simulink model "Batbot_SIM"  (Simulink 7.5)
settings: Solver=ode45  StartTime=0.0  StopTime=5  FixedStep=0.1  RelTol=1e-3
values from neighbouring files (symbols this model uses):
  F_flapping = 1000    [SimulationFB.m]
  step_2 = tf/(col-1)    [SimulationFB.m]    (also in inverse_kinematicsFULLFB.m = 0.0114285714286)
libraries: mblibv1 x76, motdrv_lib x8, simulink x7
(part 2 of 3)

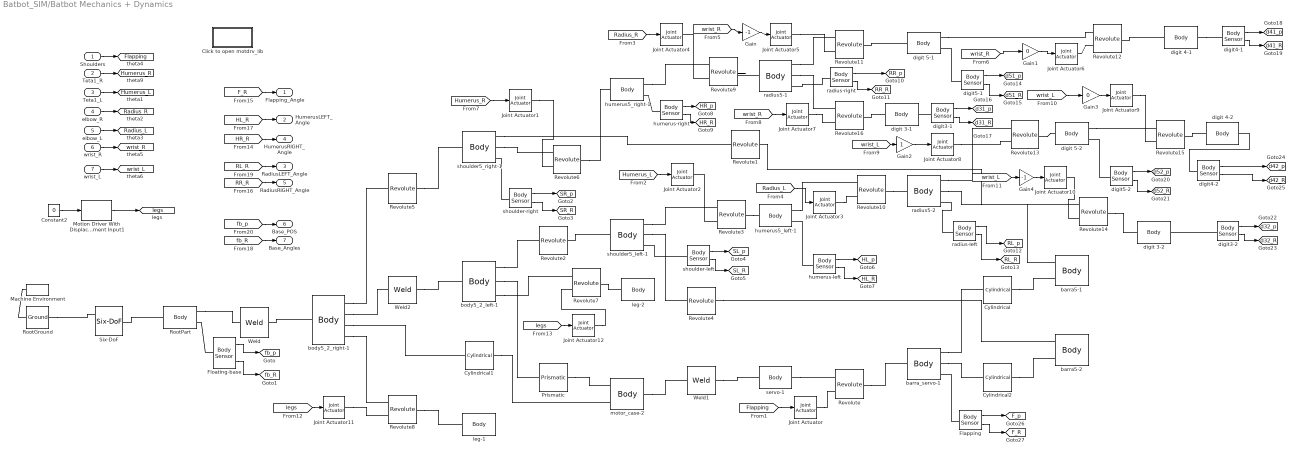
== system Batbot_SIM/Batbot Mechanics + Dynamics ==
  Shoulders : Inport  OutDataType=fixdt(1, 16)  OutScaling=2^0
  Teta1_R : Inport  Port=2  OutDataType=fixdt(1, 16)  OutScaling=2^0
  Teta1_L : Inport  Port=3  OutDataType=fixdt(1, 16)  OutScaling=2^0
  elbow_R : Inport  Port=4  OutDataType=fixdt(1, 16)  OutScaling=2^0
  elbow_L : Inport  Port=5  OutDataType=fixdt(1, 16)  OutScaling=2^0
  wrist_R : Inport  Port=6  OutDataType=fixdt(1, 16)  OutScaling=2^0
  wrist_L : Inport  Port=7  OutDataType=fixdt(1, 16)  OutScaling=2^0
  Click to open motdrv_lib : Subsystem
      settings: OpenFcn=open_system('motdrv_lib');
      mask Type: Double-click to open motdrv_lib
      mask Display: disp('motdrv_lib');
  Constant2 : Constant  Value=0  OutDataType=fixdt(1, 16)  OutScaling=2^0
  Cylindrical : mblibv1/Joints/Cylindrical  DialogController=MECH.DynMechDlgSource  PhysicalDomain=mechanical  SubClassName=Unknown  LeftPortType=blob  RightPortType=blob  LConnTagsString=__newl0  RConnTagsString=__newr0  UpdateFromCAD=on  NumSAPorts=0  CutJoint=off  MarkAsCut=off  Primitives=prismatic  PrimitiveProps=P1$WORLD$[0,0,1]$prismatic#R1$WORLD$[0,0,-1]$revolute  DialogClass=JointBlock  P1Axis=[0,0,1]  R1Axis=[0,0,-1]
  Cylindrical1 : mblibv1/Joints/Cylindrical  DialogController=MECH.DynMechDlgSource  PhysicalDomain=mechanical  SubClassName=Unknown  LeftPortType=blob  RightPortType=blob  LConnTagsString=__newl0  RConnTagsString=__newr0  UpdateFromCAD=on  NumSAPorts=0  CutJoint=off  MarkAsCut=off  Primitives=prismatic  PrimitiveProps=P1$WORLD$[0,0,-1]$prismatic#R1$WORLD$[0,0,1]$revolute  DialogClass=JointBlock  P1Axis=[0,0,-1]  R1Axis=[0,0,1]
  Cylindrical2 : mblibv1/Joints/Cylindrical  DialogController=MECH.DynMechDlgSource  PhysicalDomain=mechanical  SubClassName=Unknown  LeftPortType=blob  RightPortType=blob  LConnTagsString=__newl0  RConnTagsString=__newr0  UpdateFromCAD=on  NumSAPorts=0  CutJoint=off  MarkAsCut=off  Primitives=prismatic  PrimitiveProps=P1$WORLD$[0,0,1]$prismatic#R1$WORLD$[0,0,-1]$revolute  DialogClass=JointBlock  P1Axis=[0,0,1]  R1Axis=[0,0,-1]
  Flapping : mblibv1/Sensors &  Actuators/Body Sensor  DialogController=MECH.DynMechDlgSource  SystemSampleTime=-1  UpdateFromCAD=off  PhysicalDomain=Mechanical  PortType=blob  Muxed=off  Pose=on  Angle=on  AngleUnits=deg  ArcVelocity=off  ArcVelocityUnits=deg/s  ArcAcceleration=off  ArcAccelerationUnits=deg/s^2  CoordPosition=on  CoordPositionUnits=m  Velocity=off  VelocityUnits=m/s  Acceleration=off  AccelerationUnits=m/s^2  Quaternion=on  QuaternionDT=off  QuaternionDDT=off  QuaternionUnits=off  OutputVector=[1]  ActiveIO=on  Width=12  DialogClass=MechanicalSensorBlock  ReferenceFrame=Local (Body CS)
  Floating-base : mblibv1/Sensors &  Actuators/Body Sensor  DialogController=MECH.DynMechDlgSource  SystemSampleTime=-1  UpdateFromCAD=off  PhysicalDomain=Mechanical  PortType=blob  Muxed=off  Pose=on  Angle=on  AngleUnits=deg  ArcVelocity=off  ArcVelocityUnits=deg/s  ArcAcceleration=off  ArcAccelerationUnits=deg/s^2  CoordPosition=on  CoordPositionUnits=m  Velocity=off  VelocityUnits=m/s  Acceleration=off  AccelerationUnits=m/s^2  Quaternion=on  QuaternionDT=off  QuaternionDDT=off  QuaternionUnits=off  OutputVector=[1]  ActiveIO=on  Width=12  DialogClass=MechanicalSensorBlock  ReferenceFrame=Absolute (World)
  Gain : Gain  Gain=-1  ParameterDataType=fixdt(1, 16)  ParameterScaling=2^0  OutDataType=fixdt(1, 16)  OutScaling=2^0
  Gain1 : Gain  Gain=0  ParameterDataType=fixdt(1, 16)  ParameterScaling=2^0  OutDataType=fixdt(1, 16)  OutScaling=2^0
  Gain2 : Gain  ParameterDataType=fixdt(1, 16)  ParameterScaling=2^0  OutDataType=fixdt(1, 16)  OutScaling=2^0
  Gain3 : Gain  Gain=0  ParameterDataType=fixdt(1, 16)  ParameterScaling=2^0  OutDataType=fixdt(1, 16)  OutScaling=2^0
  Gain4 : Gain  Gain=-1  ParameterDataType=fixdt(1, 16)  ParameterScaling=2^0  OutDataType=fixdt(1, 16)  OutScaling=2^0
  Joint Actuator{,1..12} (13 alike) : mblibv1/Sensors &  Actuators/Joint Actuator  DialogController=MECH.DynMechDlgSource  SystemSampleTime=-1  UpdateFromCAD=off  PhysicalDomain=Mechanical  PortType=blob  ActuationStyle=Motion  AngleUnits=deg  ArcVelocityUnits=deg/s  ArcAccelerationUnits=deg/s^2  CoordPositionUnits=m  VelocityUnits=m/s  AccelerationUnits=m/s^2  ForceUnits=N  TorqueUnits=N*m  ActiveIO=on  Width=3  DialogClass=MechanicalActuatorBlock  Primitive=R1  ReferenceFrame=Absolute (World)
      settings: AttributesFormatString=ActuationStyle=%<ActuationStyle>
  Machine Environment : mblibv1/Bodies/Machine Environment  DialogController=MECH.DialogSource  SystemSampleTime=-1  PortType=env  PhysicalDomain=Mechanical  DialogTemplateClass=MECH.MachineEnvironment  SyncWhenCopied=off  Gravity=[0 0 0]  GravityUnits=m/s^2  GravityAsSignal=off  Dimensionality=Auto-detect  AnalysisType=Forward dynamics  LinearAssemblyTolerance=1e-3  LinearAssemblyToleranceUnits=m  AngularAssemblyTolerance=1e-3  AngularAssemblyToleranceUnits=rad  ConstraintSolverType=Stabilizing  ConstraintRelTolerance=1e-4  ConstraintAbsTolerance=1e-4  UseRobustSingularityHandling=off  RedundancyAnalysisToleranceType=Automatically select tolerance  RedundancyAnalysisTolerance=1e-14  StatePerturbationType=Fixed  PerturbationSize=1e-5  VisualizeMachine=on  BodyVisualizationType=Use model default body geometries  BodyColorSelMode=Use model default  DefaultBodyColor=[1 0 0]
  Motion Driver With Displacement Input1 : motdrv_lib/Motion Driver With Displacement Input  SystemSampleTime=-1  InitialDisplacementSource=Dialog  InitialDisplacement=0  InitialVelocity=0  TimeConstant=1e-3
  Prismatic : mblibv1/Joints/Prismatic  DialogController=MECH.DynMechDlgSource  PhysicalDomain=mechanical  SubClassName=Unknown  LeftPortType=blob  RightPortType=blob  LConnTagsString=__newl0  RConnTagsString=__newr0  UpdateFromCAD=on  NumSAPorts=0  CutJoint=off  MarkAsCut=off  Primitives=prismatic  PrimitiveProps=P1$WORLD$[-1,0,0]$prismatic  DialogClass=JointBlock  P1Axis=[-1,0,0]
  Revolute : mblibv1/Joints/Revolute  DialogController=MECH.DynMechDlgSource  PhysicalDomain=mechanical  SubClassName=Unknown  LeftPortType=blob  RightPortType=blob  LConnTagsString=__newl0|SA1  RConnTagsString=__newr0  UpdateFromCAD=on  NumSAPorts=1  CutJoint=off  MarkAsCut=off  Primitives=prismatic  PrimitiveProps=R1$Base$[0,0,-1]$revolute  DialogClass=JointBlock  R1Axis=[0,0,-1]
  Revolute1 : mblibv1/Joints/Revolute  DialogController=MECH.DynMechDlgSource  PhysicalDomain=mechanical  SubClassName=Unknown  LeftPortType=blob  RightPortType=blob  LConnTagsString=__newl0  RConnTagsString=__newr0  UpdateFromCAD=on  NumSAPorts=0  CutJoint=off  MarkAsCut=off  Primitives=prismatic  PrimitiveProps=R1$WORLD$[0,0,-1]$revolute  DialogClass=JointBlock  R1Axis=[0,0,-1]
  Revolute10 : mblibv1/Joints/Revolute  DialogController=MECH.DynMechDlgSource  PhysicalDomain=mechanical  SubClassName=Unknown  LeftPortType=blob  RightPortType=blob  LConnTagsString=__newl0|SA1  RConnTagsString=__newr0  UpdateFromCAD=on  NumSAPorts=1  CutJoint=off  MarkAsCut=off  Primitives=prismatic  PrimitiveProps=R1$Base$[0.343768,-0.939055,0]$revolute  DialogClass=JointBlock  R1Axis=[0.343768,-0.939055,0]
  Revolute11 : mblibv1/Joints/Revolute  DialogController=MECH.DynMechDlgSource  PhysicalDomain=mechanical  SubClassName=Unknown  LeftPortType=blob  RightPortType=blob  LConnTagsString=__newl0|SA1  RConnTagsString=__newr0  UpdateFromCAD=on  NumSAPorts=1  CutJoint=off  MarkAsCut=off  Primitives=prismatic  PrimitiveProps=R1$Base$[-0.399458,-0.916751,0]$revolute  DialogClass=JointBlock  R1Axis=[-0.399458,-0.916751,0]
  Revolute12 : mblibv1/Joints/Revolute  DialogController=MECH.DynMechDlgSource  PhysicalDomain=mechanical  SubClassName=Unknown  LeftPortType=blob  RightPortType=blob  LConnTagsString=__newl0|SA1  RConnTagsString=__newr0  UpdateFromCAD=on  NumSAPorts=1  CutJoint=off  MarkAsCut=off  Primitives=prismatic  PrimitiveProps=R1$Base$[0.399458,0.916751,0]$revolute  DialogClass=JointBlock  R1Axis=[0.399458,0.916751,0]
  Revolute13 : mblibv1/Joints/Revolute  DialogController=MECH.DynMechDlgSource  PhysicalDomain=mechanical  SubClassName=Unknown  LeftPortType=blob  RightPortType=blob  LConnTagsString=__newl0|SA1  RConnTagsString=__newr0  UpdateFromCAD=on  NumSAPorts=1  CutJoint=off  MarkAsCut=off  Primitives=prismatic  PrimitiveProps=R1$Base$[-0.343768,0.939055,0]$revolute  DialogClass=JointBlock  R1Axis=[-0.343768,0.939055,0]
  Revolute14 : mblibv1/Joints/Revolute  DialogController=MECH.DynMechDlgSource  PhysicalDomain=mechanical  SubClassName=Unknown  LeftPortType=blob  RightPortType=blob  LConnTagsString=__newl0|SA1  RConnTagsString=__newr0  UpdateFromCAD=on  NumSAPorts=1  CutJoint=off  MarkAsCut=off  Primitives=prismatic  PrimitiveProps=R1$Base$[0.343768,-0.939055,0]$revolute  DialogClass=JointBlock  R1Axis=[0.343768,-0.939055,0]
  Revolute15 : mblibv1/Joints/Revolute  DialogController=MECH.DynMechDlgSource  PhysicalDomain=mechanical  SubClassName=Unknown  LeftPortType=blob  RightPortType=blob  LConnTagsString=__newl0|SA1  RConnTagsString=__newr0  UpdateFromCAD=on  NumSAPorts=1  CutJoint=off  MarkAsCut=off  Primitives=prismatic  PrimitiveProps=R1$Base$[-0.343768,0.939055,0]$revolute  DialogClass=JointBlock  R1Axis=[-0.343768,0.939055,0]
  Revolute16 : mblibv1/Joints/Revolute  DialogController=MECH.DynMechDlgSource  PhysicalDomain=mechanical  SubClassName=Unknown  LeftPortType=blob  RightPortType=blob  LConnTagsString=__newl0|SA1  RConnTagsString=__newr0  UpdateFromCAD=on  NumSAPorts=1  CutJoint=off  MarkAsCut=off  Primitives=prismatic  PrimitiveProps=R1$Base$[0.399458,0.916751,0]$revolute  DialogClass=JointBlock  R1Axis=[0.399458,0.916751,0]
  Revolute2 : mblibv1/Joints/Revolute  DialogController=MECH.DynMechDlgSource  PhysicalDomain=mechanical  SubClassName=Unknown  LeftPortType=blob  RightPortType=blob  LConnTagsString=__newl0  RConnTagsString=__newr0  UpdateFromCAD=on  NumSAPorts=0  CutJoint=off  MarkAsCut=off  Primitives=prismatic  PrimitiveProps=R1$World$[0,0,-1]$revolute  DialogClass=JointBlock  R1Axis=[0,0,-1]
  Revolute3 : mblibv1/Joints/Revolute  DialogController=MECH.DynMechDlgSource  PhysicalDomain=mechanical  SubClassName=Unknown  LeftPortType=blob  RightPortType=blob  LConnTagsString=__newl0|SA1  RConnTagsString=__newr0  UpdateFromCAD=on  NumSAPorts=1  CutJoint=off  MarkAsCut=off  Primitives=prismatic  PrimitiveProps=R1$Base$[0.343768,-0.939055,0]$revolute  DialogClass=JointBlock  R1Axis=[0.343768,-0.939055,0]
  Revolute4 : mblibv1/Joints/Revolute  DialogController=MECH.DynMechDlgSource  PhysicalDomain=mechanical  SubClassName=Unknown  LeftPortType=blob  RightPortType=blob  LConnTagsString=__newl0  RConnTagsString=__newr0  UpdateFromCAD=on  NumSAPorts=0  CutJoint=off  MarkAsCut=off  Primitives=prismatic  PrimitiveProps=R1$WORLD$[0,0,-1]$revolute  DialogClass=JointBlock  R1Axis=[0,0,-1]
  Revolute5 : mblibv1/Joints/Revolute  DialogController=MECH.DynMechDlgSource  PhysicalDomain=mechanical  SubClassName=Unknown  LeftPortType=blob  RightPortType=blob  LConnTagsString=__newl0  RConnTagsString=__newr0  UpdateFromCAD=on  NumSAPorts=0  CutJoint=off  MarkAsCut=off  Primitives=prismatic  PrimitiveProps=R1$World$[0,0,1]$revolute  DialogClass=JointBlock  R1Axis=[0,0,1]
  Revolute6 : mblibv1/Joints/Revolute  DialogController=MECH.DynMechDlgSource  PhysicalDomain=mechanical  SubClassName=Unknown  LeftPortType=blob  RightPortType=blob  LConnTagsString=__newl0|SA1  RConnTagsString=__newr0  UpdateFromCAD=on  NumSAPorts=1  CutJoint=off  MarkAsCut=off  Primitives=prismatic  PrimitiveProps=R1$Base$[0.399458,0.916751,0]$revolute  DialogClass=JointBlock  R1Axis=[0.399458,0.916751,0]
  Revolute7 : mblibv1/Joints/Revolute  DialogController=MECH.DynMechDlgSource  PhysicalDomain=mechanical  SubClassName=Unknown  LeftPortType=blob  RightPortType=blob  LConnTagsString=__newl0|SA1  RConnTagsString=__newr0  UpdateFromCAD=on  NumSAPorts=1  CutJoint=off  MarkAsCut=off  Primitives=prismatic  PrimitiveProps=R1$Base$[0,1,0]$revolute  DialogClass=JointBlock  R1Axis=[0,1,0]
  Revolute8 : mblibv1/Joints/Revolute  DialogController=MECH.DynMechDlgSource  PhysicalDomain=mechanical  SubClassName=Unknown  LeftPortType=blob  RightPortType=blob  LConnTagsString=__newl0|SA1  RConnTagsString=__newr0  UpdateFromCAD=on  NumSAPorts=1  CutJoint=off  MarkAsCut=off  Primitives=prismatic  PrimitiveProps=R1$Base$[0,-1,0]$revolute  DialogClass=JointBlock  R1Axis=[0,-1,0]
  Revolute9 : mblibv1/Joints/Revolute  DialogController=MECH.DynMechDlgSource  PhysicalDomain=mechanical  SubClassName=Unknown  LeftPortType=blob  RightPortType=blob  LConnTagsString=__newl0|SA1  RConnTagsString=__newr0  UpdateFromCAD=on  NumSAPorts=1  CutJoint=off  MarkAsCut=off  Primitives=prismatic  PrimitiveProps=R1$Base$[-0.399458,-0.916751,0]$revolute  DialogClass=JointBlock  R1Axis=[-0.399458,-0.916751,0]
  RootGround : mblibv1/Bodies/Ground  DialogController=MECH.DynMechDlgSource  SystemSampleTime=-1  UpdateFromCAD=on  LeftPortType=env  RightPortType=workingframe  PhysicalDomain=Mechanical  DialogClass=GroundBlock  CoordPosition=[-0.0126203,-0.00464218,0.00877209]  CoordPositionUnits=m  StateVectorMgrId=0  MachineId=[1 0]  ShowEnvPort=on
  RootPart : mblibv1/Bodies/Body  DialogController=MECH.DynMechDlgSource  PhysicalDomain=mechanical  SubClassName=Unknown  LeftPortType=workingframe  RightPortType=workingframe  LConnTagsString=CS3  RConnTagsString=CS2|CS1  UpdateFromCAD=on  DialogClass=MechanicalBodyBlock  Mass=0  MassUnits=kg  InertiaUnits=kg*m^2  Inertia=[0,0,0;0,0,0;0,0,0]  Shape=Cylinder  ShapeDims=[1 1]  ShapeUnits=m  ShapeUse=false  Density=1  DensityUnits=kg/m^3  DensityUse=false  GraphicsMode=MACHINE_DEFAULT  BodyColorSelMode=MACHINE_DEFAULT  BodyColor=[1 0 0]  AttachedToCS=CS1  CG=Right$CG$[-0.0126203 -0.00464218 0.00877209]$WORLD$WORLD$m$[1 0 0;0 1 0;0 0 1]$3x3 Transform$rad$WORLD$false$none  WorkingFrames=Right$CS2$[0.0103788 -0.00702282 0.00503904]$WORLD$WORLD$m$[1 0 0;0 1 0;0 0 1]$3x3 Transform$rad$WORLD$true$none#Left$CS3$[-0.0126203 -0.00464218 0.00877209]$WORLD$WORLD$m$[1 0 0;0 1 0;0 0 1]$3x3 Transform$rad$WORLD$true$none#Right$CS1$[0 0 0]$WORLD$WORLD$m$[1 0 0;0 1 0;0 0 1]$3x3 Transform$rad$WORLD$true$none  CGPos=[-0.0126203 -0.00464218 0.00877209]  CGRot=[1 0 0;0 1 0;0 0 1]  CS0Pos=[]  CS0Rot=[]  CS1Pos=[0 0 0]  CS1Rot=[1 0 0;0 1 0;0 0 1]  CS2Pos=[0.0103788 -0.00702282 0.00503904]  CS2Rot=[1 0 0;0 1 0;0 0 1]  CS3Pos=[-0.0126203 -0.00464218 0.00877209]  CS3Rot=[1 0 0;0 1 0;0 0 1]  CS4Pos=[]  CS4Rot=[]  CS5Pos=[]  CS5Rot=[]  CS6Pos=[]  CS6Rot=[]  CS7Pos=[]  CS7Rot=[]  CS8Pos=[]  CS8Rot=[]  CS9Pos=[]  CS9Rot=[]  CS10Pos=[]  CS10Rot=[]  CS11Pos=[]  CS11Rot=[]  CS12Pos=[]  CS12Rot=[]  CS13Pos=[]  CS13Rot=[]  CS14Pos=[]  CS14Rot=[]  CS15Pos=[]  CS15Rot=[]  CS16Pos=[]  CS16Rot=[]  CS17Pos=[]  CS17Rot=[]  CS18Pos=[]  CS18Rot=[]  CS19Pos=[]  CS19Rot=[]  CS20Pos=[]  CS20Rot=[]
  Six-DoF : mblibv1/Joints/Six-DoF  DialogController=MECH.DynMechDlgSource  PhysicalDomain=mechanical  SubClassName=Unknown  LeftPortType=blob  RightPortType=blob  LConnTagsString=__newl0|SA1  RConnTagsString=__newr0  UpdateFromCAD=off  NumSAPorts=1  CutJoint=off  MarkAsCut=off  Primitives=prismatic_prismatic  PrimitiveProps=P1$World$[1 0 0]$prismatic#P2$World$[0 1 0]$prismatic#P3$World$[0 0 1]$prismatic#S$World$[0 0 0]$spherical  DialogClass=JointBlock  P1Axis=[1 0 0]  P2Axis=[0 1 0]  P3Axis=[0 0 1]  SAxis=[0 0 0]
  Weld : mblibv1/Joints/Weld  DialogController=MECH.DynMechDlgSource  PhysicalDomain=mechanical  SubClassName=Unknown  LeftPortType=blob  RightPortType=blob  LConnTagsString=__newl0  RConnTagsString=__newr0  UpdateFromCAD=on  NumSAPorts=0  CutJoint=off  MarkAsCut=off  Primitives=weld  PrimitiveProps=W$World$[0.57735,0.57735,0.57735]$weld  DialogClass=JointBlock  WAxis=[0.57735,0.57735,0.57735]
  Weld1 : mblibv1/Joints/Weld  DialogController=MECH.DynMechDlgSource  PhysicalDomain=mechanical  SubClassName=Unknown  LeftPortType=blob  RightPortType=blob  LConnTagsString=__newl0  RConnTagsString=__newr0  UpdateFromCAD=on  NumSAPorts=0  CutJoint=off  MarkAsCut=off  Primitives=weld  PrimitiveProps=W$WORLD$[0.57735,0.57735,0.57735]$weld  DialogClass=JointBlock  WAxis=[0.57735,0.57735,0.57735]
  Weld2 : mblibv1/Joints/Weld  DialogController=MECH.DynMechDlgSource  PhysicalDomain=mechanical  SubClassName=Unknown  LeftPortType=blob  RightPortType=blob  LConnTagsString=__newl0  RConnTagsString=__newr0  UpdateFromCAD=on  NumSAPorts=0  CutJoint=off  MarkAsCut=off  Primitives=weld  PrimitiveProps=W$WORLD$[0.57735,0.57735,0.57735]$weld  DialogClass=JointBlock  WAxis=[0.57735,0.57735,0.57735]
  barra5-1 : mblibv1/Bodies/Body  DialogController=MECH.DynMechDlgSource  PhysicalDomain=mechanical  SubClassName=Unknown  LeftPortType=workingframe  RightPortType=workingframe  LConnTagsString=CS2|CS3  UpdateFromCAD=on  DialogClass=MechanicalBodyBlock  Mass=0.000119962  MassUnits=kg  InertiaUnits=kg*m^2  Inertia=[1.1412e-010,-3.7491e-012,4.37309e-017;-3.7491e-012,8.63077e-009,-5.97977e-019;4.37309e-017,-5.97977e-019,8.66519e-009]  Shape=Cylinder  ShapeDims=[1 1]  ShapeUnits=m  ShapeUse=false  Density=1  DensityUnits=kg/m^3  DensityUse=false  GraphicsMode=GFXFILE  GraphicsFileName=Batbot - barra5-1.STL  BodyColorSelMode=COLORPALETTE  BodyColor=[0.25098 0.25098 0.25098]  AttachedToCS=CS1  CG=Right$CG$[0.00675046 0.021022 0.006]$WORLD$WORLD$m$[0.97857 0.205912 0;-0.205912 0.97857 0;0 0 1]$3x3 Transform$rad$WORLD$false$none  WorkingFrames=Right$CS1$[-0.00713958 0.0218999 0.007]$WORLD$WORLD$m$[0.97857 0.205912 0;-0.205912 0.97857 0;0 0 1]$3x3 Transform$rad$WORLD$false$none#Left$CS2$[0.0201957 0.0181917 0.005]$WORLD$WORLD$m$[1 0 0;0 1 0;0 0 1]$3x3 Transform$rad$WORLD$true$none#Left$CS3$[-0.00672776 0.023857 0.005]$WORLD$WORLD$m$[1 0 0;0 1 0;0 0 1]$3x3 Transform$rad$WORLD$true$none#Right$CS4$[0 0 0]$WORLD$WORLD$m$[1 0 0;0 1 0;0 0 1]$3x3 Transform$rad$WORLD$false$none  CGPos=[0.00675046 0.021022 0.006]  CGRot=[0.97857 0.205912 0;-0.205912 0.97857 0;0 0 1]  CS0Pos=[]  CS0Rot=[]  CS1Pos=[-0.00713958 0.0218999 0.007]  CS1Rot=[0.97857 0.205912 0;-0.205912 0.97857 0;0 0 1]  CS2Pos=[0.0201957 0.0181917 0.005]  CS2Rot=[1 0 0;0 1 0;0 0 1]  CS3Pos=[-0.00672776 0.023857 0.005]  CS3Rot=[1 0 0;0 1 0;0 0 1]  CS4Pos=[0 0 0]  CS4Rot=[1 0 0;0 1 0;0 0 1]  CS5Pos=[]  CS5Rot=[]  CS6Pos=[]  CS6Rot=[]  CS7Pos=[]  CS7Rot=[]  CS8Pos=[]  CS8Rot=[]  CS9Pos=[]  CS9Rot=[]  CS10Pos=[]  CS10Rot=[]  CS11Pos=[]  CS11Rot=[]  CS12Pos=[]  CS12Rot=[]  CS13Pos=[]  CS13Rot=[]  CS14Pos=[]  CS14Rot=[]  CS15Pos=[]  CS15Rot=[]  CS16Pos=[]  CS16Rot=[]  CS17Pos=[]  CS17Rot=[]  CS18Pos=[]  CS18Rot=[]  CS19Pos=[]  CS19Rot=[]  CS20Pos=[]  CS20Rot=[]
  barra5-2 : mblibv1/Bodies/Body  DialogController=MECH.DynMechDlgSource  PhysicalDomain=mechanical  SubClassName=Unknown  LeftPortType=workingframe  RightPortType=workingframe  LConnTagsString=CS2|CS3  UpdateFromCAD=on  DialogClass=MechanicalBodyBlock  Mass=0.000119962  MassUnits=kg  InertiaUnits=kg*m^2  Inertia=[1.1412e-010,-3.7491e-012,4.37309e-017;-3.7491e-012,8.63077e-009,-5.97977e-019;4.37309e-017,-5.97977e-019,8.66519e-009]  Shape=Cylinder  ShapeDims=[1 1]  ShapeUnits=m  ShapeUse=false  Density=1  DensityUnits=kg/m^3  DensityUse=false  GraphicsMode=GFXFILE  GraphicsFileName=Batbot - barra5-2.STL  BodyColorSelMode=COLORPALETTE  BodyColor=[0.25098;0.25098;0.25098]  AttachedToCS=CS1  CG=Right$CG$[-0.0314187 0.0149284 0.006]$WORLD$WORLD$m$[0.96422 0.265104 0;-0.265104 0.96422 0;0 0 1]$3x3 Transform$rad$WORLD$false$none  WorkingFrames=Right$CS1$[-0.0452295 0.0166503 0.007]$WORLD$WORLD$m$[0.96422 0.265104 0;-0.265104 0.96422 0;0 0 1]$3x3 Transform$rad$WORLD$false$none#Left$CS2$[-0.0446993 0.0185787 0.005]$WORLD$WORLD$m$[1 0 0;0 1 0;0 0 1]$3x3 Transform$rad$WORLD$true$none#Left$CS3$[-0.0181707 0.0112849 0.005]$WORLD$WORLD$m$[1 0 0;0 1 0;0 0 1]$3x3 Transform$rad$WORLD$true$none  CGPos=[-0.0314187 0.0149284 0.006]  CGRot=[0.96422 0.265104 0;-0.265104 0.96422 0;0 0 1]  CS0Pos=[]  CS0Rot=[]  CS1Pos=[-0.0452295 0.0166503 0.007]  CS1Rot=[0.96422 0.265104 0;-0.265104 0.96422 0;0 0 1]  CS2Pos=[-0.0446993 0.0185787 0.005]  CS2Rot=[1 0 0;0 1 0;0 0 1]  CS3Pos=[-0.0181707 0.0112849 0.005]  CS3Rot=[1 0 0;0 1 0;0 0 1]  CS4Pos=[]  CS4Rot=[]  CS5Pos=[]  CS5Rot=[]  CS6Pos=[]  CS6Rot=[]  CS7Pos=[]  CS7Rot=[]  CS8Pos=[]  CS8Rot=[]  CS9Pos=[]  CS9Rot=[]  CS10Pos=[]  CS10Rot=[]  CS11Pos=[]  CS11Rot=[]  CS12Pos=[]  CS12Rot=[]  CS13Pos=[]  CS13Rot=[]  CS14Pos=[]  CS14Rot=[]  CS15Pos=[]  CS15Rot=[]  CS16Pos=[]  CS16Rot=[]  CS17Pos=[]  CS17Rot=[]  CS18Pos=[]  CS18Rot=[]  CS19Pos=[]  CS19Rot=[]  CS20Pos=[]  CS20Rot=[]
  barra_servo-1 : mblibv1/Bodies/Body  DialogController=MECH.DynMechDlgSource  PhysicalDomain=mechanical  SubClassName=Unknown  LeftPortType=workingframe  RightPortType=workingframe  LConnTagsString=CS2  RConnTagsString=CS3|CS4|CS5  UpdateFromCAD=on  DialogClass=MechanicalBodyBlock  Mass=0.00014427  MassUnits=kg  InertiaUnits=kg*m^2  Inertia=[7.38605e-009,0,0;0,7.70092e-009,0;0,0,5.0296e-010]  Shape=Cylinder  ShapeDims=[1 1]  ShapeUnits=m  ShapeUse=false  Density=1  DensityUnits=kg/m^3  DensityUse=false  GraphicsMode=GFXFILE  GraphicsFileName=Batbot - barra_servo-1.STL  BodyColorSelMode=COLORPALETTE  BodyColor=[1 1 1]  AttachedToCS=CS1  CG=Right$CG$[-0.0124493 0.017571 0.00472003]$WORLD$WORLD$m$[-0.739536 0 -0.673117;0.673117 0 -0.739536;0 -1 0]$3x3 Transform$rad$WORLD$false$none  WorkingFrames=Right$CS1$[-0.0124493 0.017571 0.0095]$WORLD$WORLD$m$[-0.739536 0 -0.673117;0.673117 0 -0.739536;0 -1 0]$3x3 Transform$rad$WORLD$false$none#Left$CS2$[-0.0124493 0.017571 0.0095]$WORLD$WORLD$m$[1 0 0;0 1 0;0 0 1]$3x3 Transform$rad$WORLD$true$none#Right$CS3$[-0.00672776 0.023857 0.005]$WORLD$WORLD$m$[1 0 0;0 1 0;0 0 1]$3x3 Transform$rad$WORLD$true$none#Right$CS4$[-0.0181707 0.0112849 0.005]$WORLD$WORLD$m$[1 0 0;0 1 0;0 0 1]$3x3 Transform$rad$WORLD$true$none#Right$CS5$[0 0 0]$WORLD$WORLD$m$[1 0 0;0 1 0;0 0 1]$3x3 Transform$rad$WORLD$true$none  CGPos=[-0.0124493 0.017571 0.00472003]  CGRot=[-0.739536 0 -0.673117;0.673117 0 -0.739536;0 -1 0]  CS0Pos=[]  CS0Rot=[]  CS1Pos=[-0.0124493 0.017571 0.0095]  CS1Rot=[-0.739536 0 -0.673117;0.673117 0 -0.739536;0 -1 0]  CS2Pos=[-0.0124493 0.017571 0.0095]  CS2Rot=[1 0 0;0 1 0;0 0 1]  CS3Pos=[-0.00672776 0.023857 0.005]  CS3Rot=[1 0 0;0 1 0;0 0 1]  CS4Pos=[-0.0181707 0.0112849 0.005]  CS4Rot=[1 0 0;0 1 0;0 0 1]  CS5Pos=[0 0 0]  CS5Rot=[1 0 0;0 1 0;0 0 1]  CS6Pos=[]  CS6Rot=[]  CS7Pos=[]  CS7Rot=[]  CS8Pos=[]  CS8Rot=[]  CS9Pos=[]  CS9Rot=[]  CS10Pos=[]  CS10Rot=[]  CS11Pos=[]  CS11Rot=[]  CS12Pos=[]  CS12Rot=[]  CS13Pos=[]  CS13Rot=[]  CS14Pos=[]  CS14Rot=[]  CS15Pos=[]  CS15Rot=[]  CS16Pos=[]  CS16Rot=[]  CS17Pos=[]  CS17Rot=[]  CS18Pos=[]  CS18Rot=[]  CS19Pos=[]  CS19Rot=[]  CS20Pos=[]  CS20Rot=[]
  body5_2_left-1 : mblibv1/Bodies/Body  DialogController=MECH.DynMechDlgSource  PhysicalDomain=mechanical  SubClassName=Unknown  LeftPortType=workingframe  RightPortType=workingframe  LConnTagsString=CS3  RConnTagsString=CS2|CS4|CS5  UpdateFromCAD=on  DialogClass=MechanicalBodyBlock  Mass=0.00990124  MassUnits=kg  InertiaUnits=kg*m^2  Inertia=[6.86716e-006,1.97503e-007,-1.60321e-007;1.97503e-007,6.52126e-006,2.23269e-008;-1.60321e-007,2.23269e-008,1.26887e-006]  Shape=Cylinder  ShapeDims=[1 1]  ShapeUnits=m  ShapeUse=false  Density=1  DensityUnits=kg/m^3  DensityUse=false  GraphicsMode=GFXFILE  GraphicsFileName=Batbot - body5_2_left-1.STL  BodyColorSelMode=COLORPALETTE  BodyColor=[0.25098;0.25098;0.25098]  AttachedToCS=CS1  CG=Right$CG$[-0.0358488 -0.00702322 0.00503721]$WORLD$WORLD$m$[1 0 0;0 1 0;0 0 1]$3x3 Transform$rad$WORLD$false$none  WorkingFrames=Right$CS1$[0.00126505 0.00228611 -2.18436e-014]$WORLD$WORLD$m$[1 0 0;0 1 0;0 0 1]$3x3 Transform$rad$WORLD$false$none#Right$CS2$[-0.0387349 0.00228611 0.034]$WORLD$WORLD$m$[1 0 0;0 1 0;0 0 1]$3x3 Transform$rad$WORLD$true$none#Left$CS3$[-0.0127349 -0.0177139 0.035]$WORLD$WORLD$m$[1 0 0;0 1 0;0 0 1]$3x3 Transform$rad$WORLD$true$none#Right$CS4$[-0.0127349 -0.0167139 0.019]$WORLD$WORLD$m$[1 0 0;0 1 0;0 0 1]$3x3 Transform$rad$WORLD$true$none#Right$CS5$[-0.0367349 0.00438611 0.052]$WORLD$WORLD$m$[1 0 0;0 1 0;0 0 1]$3x3 Transform$rad$WORLD$true$none  CGPos=[-0.0358488 -0.00702322 0.00503721]  CGRot=[1 0 0;0 1 0;0 0 1]  CS0Pos=[]  CS0Rot=[]  CS1Pos=[0.00126505 0.00228611 -2.18436e-014]  CS1Rot=[1 0 0;0 1 0;0 0 1]  CS2Pos=[-0.0387349 0.00228611 0.034]  CS2Rot=[1 0 0;0 1 0;0 0 1]  CS3Pos=[-0.0127349 -0.0177139 0.035]  CS3Rot=[1 0 0;0 1 0;0 0 1]  CS4Pos=[-0.0127349 -0.0167139 0.019]  CS4Rot=[1 0 0;0 1 0;0 0 1]  CS5Pos=[-0.0367349 0.00438611 0.052]  CS5Rot=[1 0 0;0 1 0;0 0 1]  CS6Pos=[]  CS6Rot=[]  CS7Pos=[]  CS7Rot=[]  CS8Pos=[]  CS8Rot=[]  CS9Pos=[]  CS9Rot=[]  CS10Pos=[]  CS10Rot=[]  CS11Pos=[]  CS11Rot=[]  CS12Pos=[]  CS12Rot=[]  CS13Pos=[]  CS13Rot=[]  CS14Pos=[]  CS14Rot=[]  CS15Pos=[]  CS15Rot=[]  CS16Pos=[]  CS16Rot=[]  CS17Pos=[]  CS17Rot=[]  CS18Pos=[]  CS18Rot=[]  CS19Pos=[]  CS19Rot=[]  CS20Pos=[]  CS20Rot=[]
  body5_2_right-1 : mblibv1/Bodies/Body  DialogController=MECH.DynMechDlgSource  PhysicalDomain=mechanical  SubClassName=Unknown  LeftPortType=workingframe  RightPortType=workingframe  LConnTagsString=CS2  RConnTagsString=CS3|CS4|CS5|CS6  UpdateFromCAD=on  DialogClass=MechanicalBodyBlock  Mass=0.00990077  MassUnits=kg  InertiaUnits=kg*m^2  Inertia=[6.8671e-006,-1.97521e-007,1.60303e-007;-1.97521e-007,6.52112e-006,2.23345e-008;1.60303e-007,2.23345e-008,1.26891e-006]  Shape=Cylinder  ShapeDims=[1 1]  ShapeUnits=m  ShapeUse=false  Density=1  DensityUnits=kg/m^3  DensityUse=false  GraphicsMode=GFXFILE  GraphicsFileName=Batbot - body5_2_right-1.STL  BodyColorSelMode=COLORPALETTE  BodyColor=[0.25098;0.25098;0.25098]  AttachedToCS=CS1  CG=Right$CG$[0.0103788 -0.00702282 0.00503904]$WORLD$WORLD$m$[1 0 0;0 1 0;0 0 1]$3x3 Transform$rad$WORLD$false$none  WorkingFrames=Right$CS1$[0.00126505 0.00228611 -2.18402e-014]$WORLD$WORLD$m$[1 0 0;0 1 0;0 0 1]$3x3 Transform$rad$WORLD$false$none#Left$CS2$[0.0103788 -0.00702282 0.00503904]$WORLD$WORLD$m$[1 0 0;0 1 0;0 0 1]$3x3 Transform$rad$WORLD$true$none#Right$CS3$[0.0132651 0.00228611 0.034]$WORLD$WORLD$m$[1 0 0;0 1 0;0 0 1]$3x3 Transform$rad$WORLD$true$none#Right$CS4$[-0.0127349 -0.0177139 0.035]$WORLD$WORLD$m$[1 0 0;0 1 0;0 0 1]$3x3 Transform$rad$WORLD$true$none#Right$CS5$[-0.00498495 -0.0167139 0.019]$WORLD$WORLD$m$[1 0 0;0 1 0;0 0 1]$3x3 Transform$rad$WORLD$true$none#Right$CS6$[0.0112651 0.00438611 0.052]$WORLD$WORLD$m$[1 0 0;0 1 0;0 0 1]$3x3 Transform$rad$WORLD$true$none  CGPos=[0.0103788 -0.00702282 0.00503904]  CGRot=[1 0 0;0 1 0;0 0 1]  CS0Pos=[]  CS0Rot=[]  CS1Pos=[0.00126505 0.00228611 -2.18402e-014]  CS1Rot=[1 0 0;0 1 0;0 0 1]  CS2Pos=[0.0103788 -0.00702282 0.00503904]  CS2Rot=[1 0 0;0 1 0;0 0 1]  CS3Pos=[0.0132651 0.00228611 0.034]  CS3Rot=[1 0 0;0 1 0;0 0 1]  CS4Pos=[-0.0127349 -0.0177139 0.035]  CS4Rot=[1 0 0;0 1 0;0 0 1]  CS5Pos=[-0.00498495 -0.0167139 0.019]  CS5Rot=[1 0 0;0 1 0;0 0 1]  CS6Pos=[0.0112651 0.00438611 0.052]  CS6Rot=[1 0 0;0 1 0;0 0 1]  CS7Pos=[]  CS7Rot=[]  CS8Pos=[]  CS8Rot=[]  CS9Pos=[]  CS9Rot=[]  CS10Pos=[]  CS10Rot=[]  CS11Pos=[]  CS11Rot=[]  CS12Pos=[]  CS12Rot=[]  CS13Pos=[]  CS13Rot=[]  CS14Pos=[]  CS14Rot=[]  CS15Pos=[]  CS15Rot=[]  CS16Pos=[]  CS16Rot=[]  CS17Pos=[]  CS17Rot=[]  CS18Pos=[]  CS18Rot=[]  CS19Pos=[]  CS19Rot=[]  CS20Pos=[]  CS20Rot=[]
  digit 3-1 : mblibv1/Bodies/Body  DialogController=MECH.DynMechDlgSource  PhysicalDomain=mechanical  SubClassName=Unknown  LeftPortType=workingframe  RightPortType=workingframe  LConnTagsString=CS2  RConnTagsString=CS3  UpdateFromCAD=on  DialogClass=MechanicalBodyBlock  Mass=0.000927477  MassUnits=kg  InertiaUnits=kg*m^2  Inertia=[4.25859e-008,5.30437e-013,-1.56119e-007;5.30437e-013,9.99762e-007,1.56782e-013;-1.56119e-007,1.56782e-013,9.57517e-007]  Shape=Cylinder  ShapeDims=[1 1]  ShapeUnits=m  ShapeUse=false  Density=1  DensityUnits=kg/m^3  DensityUse=false  GraphicsMode=GFXFILE  GraphicsFileName=Batbot - digit 3-1.STL  BodyColorSelMode=COLORPALETTE  BodyColor=[0.25098 0.25098 0.25098]  AttachedToCS=CS1  CG=Right$CG$[0.133076 -0.047356 -0.0341214]$WORLD$WORLD$m$[0.916713 0.399458 0.0083752;-0.399442 0.916751 -0.00364935;-0.00913574 0 0.999958]$3x3 Transform$rad$WORLD$false$none  WorkingFrames=Right$CS1$[0.0990975 -0.0333686 -0.0365888]$WORLD$WORLD$m$[0.916713 0.399458 0.0083752;-0.399442 0.916751 -0.00364935;-0.00913574 0 0.999958]$3x3 Transform$rad$WORLD$false$none#Left$CS2$[0.0996967 -0.0319935 -0.0365888]$WORLD$WORLD$m$[1 0 0;0 1 0;0 0 1]$3x3 Transform$rad$WORLD$true$none#Right$CS3$[0 0 0]$WORLD$WORLD$m$[1 0 0;0 1 0;0 0 1]$3x3 Transform$rad$WORLD$true$none  CGPos=[0.133076 -0.047356 -0.0341214]  CGRot=[0.916713 0.399458 0.0083752;-0.399442 0.916751 -0.00364935;-0.00913574 0 0.999958]  CS0Pos=[]  CS0Rot=[]  CS1Pos=[0.0990975 -0.0333686 -0.0365888]  CS1Rot=[0.916713 0.399458 0.0083752;-0.399442 0.916751 -0.00364935;-0.00913574 0 0.999958]  CS2Pos=[0.0996967 -0.0319935 -0.0365888]  CS2Rot=[1 0 0;0 1 0;0 0 1]  CS3Pos=[0 0 0]  CS3Rot=[1 0 0;0 1 0;0 0 1]  CS4Pos=[]  CS4Rot=[]  CS5Pos=[]  CS5Rot=[]  CS6Pos=[]  CS6Rot=[]  CS7Pos=[]  CS7Rot=[]  CS8Pos=[]  CS8Rot=[]  CS9Pos=[]  CS9Rot=[]  CS10Pos=[]  CS10Rot=[]  CS11Pos=[]  CS11Rot=[]  CS12Pos=[]  CS12Rot=[]  CS13Pos=[]  CS13Rot=[]  CS14Pos=[]  CS14Rot=[]  CS15Pos=[]  CS15Rot=[]  CS16Pos=[]  CS16Rot=[]  CS17Pos=[]  CS17Rot=[]  CS18Pos=[]  CS18Rot=[]  CS19Pos=[]  CS19Rot=[]  CS20Pos=[]  CS20Rot=[]
  digit 3-2 : mblibv1/Bodies/Body  DialogController=MECH.DynMechDlgSource  PhysicalDomain=mechanical  SubClassName=Unknown  LeftPortType=workingframe  RightPortType=workingframe  LConnTagsString=CS2  RConnTagsString=CS3  UpdateFromCAD=on  DialogClass=MechanicalBodyBlock  Mass=0.000927477  MassUnits=kg  InertiaUnits=kg*m^2  Inertia=[4.25859e-008,5.30437e-013,-1.56119e-007;5.30437e-013,9.99762e-007,1.56782e-013;-1.56119e-007,1.56782e-013,9.57517e-007]  Shape=Cylinder  ShapeDims=[1 1]  ShapeUnits=m  ShapeUse=false  Density=1  DensityUnits=kg/m^3  DensityUse=false  GraphicsMode=GFXFILE  GraphicsFileName=Batbot - digit 3-2.STL  BodyColorSelMode=COLORPALETTE  BodyColor=[0.25098 0.25098 0.25098]  AttachedToCS=CS1  CG=Right$CG$[-0.159324 -0.0438292 -0.0110989]$WORLD$WORLD$m$[-0.911682 0.343768 0.225077;-0.333748 -0.939054 0.0823959;0.239684 0 0.970851]$3x3 Transform$rad$WORLD$false$none  WorkingFrames=Right$CS1$[-0.126742 -0.0311028 -0.0226197]$WORLD$WORLD$m$[-0.911682 0.343768 0.225077;-0.333748 -0.939054 0.0823959;0.239684 0 0.970851]$3x3 Transform$rad$WORLD$false$none#Left$CS2$[-0.126226 -0.0325114 -0.0226197]$WORLD$WORLD$m$[1 0 0;0 1 0;0 0 1]$3x3 Transform$rad$WORLD$true$none#Right$CS3$[0 0 0]$WORLD$WORLD$m$[1 0 0;0 1 0;0 0 1]$3x3 Transform$rad$WORLD$true$none  CGPos=[-0.159324 -0.0438292 -0.0110989]  CGRot=[-0.911682 0.343768 0.225077;-0.333748 -0.939054 0.0823959;0.239684 0 0.970851]  CS0Pos=[]  CS0Rot=[]  CS1Pos=[-0.126742 -0.0311028 -0.0226197]  CS1Rot=[-0.911682 0.343768 0.225077;-0.333748 -0.939054 0.0823959;0.239684 0 0.970851]  CS2Pos=[-0.126226 -0.0325114 -0.0226197]  CS2Rot=[1 0 0;0 1 0;0 0 1]  CS3Pos=[0 0 0]  CS3Rot=[1 0 0;0 1 0;0 0 1]  CS4Pos=[]  CS4Rot=[]  CS5Pos=[]  CS5Rot=[]  CS6Pos=[]  CS6Rot=[]  CS7Pos=[]  CS7Rot=[]  CS8Pos=[]  CS8Rot=[]  CS9Pos=[]  CS9Rot=[]  CS10Pos=[]  CS10Rot=[]  CS11Pos=[]  CS11Rot=[]  CS12Pos=[]  CS12Rot=[]  CS13Pos=[]  CS13Rot=[]  CS14Pos=[]  CS14Rot=[]  CS15Pos=[]  CS15Rot=[]  CS16Pos=[]  CS16Rot=[]  CS17Pos=[]  CS17Rot=[]  CS18Pos=[]  CS18Rot=[]  CS19Pos=[]  CS19Rot=[]  CS20Pos=[]  CS20Rot=[]
  digit 4-1 : mblibv1/Bodies/Body  DialogController=MECH.DynMechDlgSource  PhysicalDomain=mechanical  SubClassName=Unknown  LeftPortType=workingframe  RightPortType=workingframe  LConnTagsString=CS2  RConnTagsString=CS3  UpdateFromCAD=on  DialogClass=MechanicalBodyBlock  Mass=0.000580341  MassUnits=kg  InertiaUnits=kg*m^2  Inertia=[3.08423e-009,6.78726e-009,-1.17599e-008;6.78726e-009,4.86668e-007,2.38134e-010;-1.17599e-008,2.38134e-010,4.84021e-007]  Shape=Cylinder  ShapeDims=[1 1]  ShapeUnits=m  ShapeUse=false  Density=1  DensityUnits=kg/m^3  DensityUse=false  GraphicsMode=GFXFILE  GraphicsFileName=Batbot - digit 4-1.STL  BodyColorSelMode=COLORPALETTE  BodyColor=[0.25098 0.25098 0.25098]  AttachedToCS=CS1  CG=Right$CG$[0.122562 -0.0453793 -0.0240151]$WORLD$WORLD$m$[0.832482 0.399458 -0.383936;-0.362739 0.916751 0.167293;0.418801 0 0.908078]$3x3 Transform$rad$WORLD$false$none  WorkingFrames=Right$CS1$[0.0974597 -0.0371273 -0.0365888]$WORLD$WORLD$m$[0.832482 0.399458 -0.383936;-0.362739 0.916751 0.167293;0.418801 0 0.908078]$3x3 Transform$rad$WORLD$false$none#Left$CS2$[0.0982587 -0.0352938 -0.0365888]$WORLD$WORLD$m$[1 0 0;0 1 0;0 0 1]$3x3 Transform$rad$WORLD$true$none#Right$CS3$[0 0 0]$WORLD$WORLD$m$[1 0 0;0 1 0;0 0 1]$3x3 Transform$rad$WORLD$true$none  CGPos=[0.122562 -0.0453793 -0.0240151]  CGRot=[0.832482 0.399458 -0.383936;-0.362739 0.916751 0.167293;0.418801 0 0.908078]  CS0Pos=[]  CS0Rot=[]  CS1Pos=[0.0974597 -0.0371273 -0.0365888]  CS1Rot=[0.832482 0.399458 -0.383936;-0.362739 0.916751 0.167293;0.418801 0 0.908078]  CS2Pos=[0.0982587 -0.0352938 -0.0365888]  CS2Rot=[1 0 0;0 1 0;0 0 1]  CS3Pos=[0 0 0]  CS3Rot=[1 0 0;0 1 0;0 0 1]  CS4Pos=[]  CS4Rot=[]  CS5Pos=[]  CS5Rot=[]  CS6Pos=[]  CS6Rot=[]  CS7Pos=[]  CS7Rot=[]  CS8Pos=[]  CS8Rot=[]  CS9Pos=[]  CS9Rot=[]  CS10Pos=[]  CS10Rot=[]  CS11Pos=[]  CS11Rot=[]  CS12Pos=[]  CS12Rot=[]  CS13Pos=[]  CS13Rot=[]  CS14Pos=[]  CS14Rot=[]  CS15Pos=[]  CS15Rot=[]  CS16Pos=[]  CS16Rot=[]  CS17Pos=[]  CS17Rot=[]  CS18Pos=[]  CS18Rot=[]  CS19Pos=[]  CS19Rot=[]  CS20Pos=[]  CS20Rot=[]
  digit 4-2 : mblibv1/Bodies/Body  DialogController=MECH.DynMechDlgSource  PhysicalDomain=mechanical  SubClassName=Unknown  LeftPortType=workingframe  RightPortType=workingframe  LConnTagsString=CS2  RConnTagsString=CS3  UpdateFromCAD=on  DialogClass=MechanicalBodyBlock  Mass=0.000580341  MassUnits=kg  InertiaUnits=kg*m^2  Inertia=[3.08423e-009,6.78726e-009,-1.17599e-008;6.78726e-009,4.86668e-007,2.38134e-010;-1.17599e-008,2.38134e-010,4.84021e-007]  Shape=Cylinder  ShapeDims=[1 1]  ShapeUnits=m  ShapeUse=false  Density=1  DensityUnits=kg/m^3  DensityUse=false  GraphicsMode=GFXFILE  GraphicsFileName=Batbot - digit 4-2.STL  BodyColorSelMode=COLORPALETTE  BodyColor=[0.25098 0.25098 0.25098]  AttachedToCS=CS1  CG=Right$CG$[-0.146347 -0.0365357 -0.00166556]$WORLD$WORLD$m$[-0.662216 0.343768 0.665803;-0.242424 -0.939054 0.243736;0.709014 0 0.705195]$3x3 Transform$rad$WORLD$false$none  WorkingFrames=Right$CS1$[-0.128151 -0.0272527 -0.0226197]$WORLD$WORLD$m$[-0.662216 0.343768 0.665803;-0.242424 -0.939054 0.243736;0.709014 0 0.705195]$3x3 Transform$rad$WORLD$false$none#Left$CS2$[-0.127464 -0.0291308 -0.0226197]$WORLD$WORLD$m$[1 0 0;0 1 0;0 0 1]$3x3 Transform$rad$WORLD$true$none#Right$CS3$[0 0 0]$WORLD$WORLD$m$[1 0 0;0 1 0;0 0 1]$3x3 Transform$rad$WORLD$true$none  CGPos=[-0.146347 -0.0365357 -0.00166556]  CGRot=[-0.662216 0.343768 0.665803;-0.242424 -0.939054 0.243736;0.709014 0 0.705195]  CS0Pos=[]  CS0Rot=[]  CS1Pos=[-0.128151 -0.0272527 -0.0226197]  CS1Rot=[-0.662216 0.343768 0.665803;-0.242424 -0.939054 0.243736;0.709014 0 0.705195]  CS2Pos=[-0.127464 -0.0291308 -0.0226197]  CS2Rot=[1 0 0;0 1 0;0 0 1]  CS3Pos=[0 0 0]  CS3Rot=[1 0 0;0 1 0;0 0 1]  CS4Pos=[]  CS4Rot=[]  CS5Pos=[]  CS5Rot=[]  CS6Pos=[]  CS6Rot=[]  CS7Pos=[]  CS7Rot=[]  CS8Pos=[]  CS8Rot=[]  CS9Pos=[]  CS9Rot=[]  CS10Pos=[]  CS10Rot=[]  CS11Pos=[]  CS11Rot=[]  CS12Pos=[]  CS12Rot=[]  CS13Pos=[]  CS13Rot=[]  CS14Pos=[]  CS14Rot=[]  CS15Pos=[]  CS15Rot=[]  CS16Pos=[]  CS16Rot=[]  CS17Pos=[]  CS17Rot=[]  CS18Pos=[]  CS18Rot=[]  CS19Pos=[]  CS19Rot=[]  CS20Pos=[]  CS20Rot=[]
  digit 5-1 : mblibv1/Bodies/Body  DialogController=MECH.DynMechDlgSource  PhysicalDomain=mechanical  SubClassName=Unknown  LeftPortType=workingframe  RightPortType=workingframe  LConnTagsString=CS2  RConnTagsString=CS3|CS4  UpdateFromCAD=on  DialogClass=MechanicalBodyBlock  Mass=0.000627913  MassUnits=kg  InertiaUnits=kg*m^2  Inertia=[4.77978e-009,7.52312e-009,6.57727e-010;7.52312e-009,4.69347e-007,-6.68752e-011;6.57727e-010,-6.68752e-011,4.65325e-007]  Shape=Cylinder  ShapeDims=[1 1]  ShapeUnits=m  ShapeUse=false  Density=1  DensityUnits=kg/m^3  DensityUse=false  GraphicsMode=GFXFILE  GraphicsFileName=Batbot - digit 5-1.STL  BodyColorSelMode=COLORPALETTE  BodyColor=[0.25098 0.25098 0.25098]  AttachedToCS=CS1  CG=Right$CG$[0.10572 -0.0398072 -0.0236482]$WORLD$WORLD$m$[0.499609 0.399458 -0.768651;-0.217696 0.916751 0.334926;0.838451 0 0.544978]$3x3 Transform$rad$WORLD$false$none  WorkingFrames=Right$CS1$[0.0966608 -0.0389608 -0.0365888]$WORLD$WORLD$m$[0.499609 0.399458 -0.768651;-0.217696 0.916751 0.334926;0.838451 0 0.544978]$3x3 Transform$rad$WORLD$false$none#Left$CS2$[0.0976595 -0.0366689 -0.0365888]$WORLD$WORLD$m$[1 0 0;0 1 0;0 0 1]$3x3 Transform$rad$WORLD$true$none#Right$CS3$[0.0982587 -0.0352938 -0.0365888]$WORLD$WORLD$m$[1 0 0;0 1 0;0 0 1]$3x3 Transform$rad$WORLD$true$none#Right$CS4$[0 0 0]$WORLD$WORLD$m$[1 0 0;0 1 0;0 0 1]$3x3 Transform$rad$WORLD$true$none  CGPos=[0.10572 -0.0398072 -0.0236482]  CGRot=[0.499609 0.399458 -0.768651;-0.217696 0.916751 0.334926;0.838451 0 0.544978]  CS0Pos=[]  CS0Rot=[]  CS1Pos=[0.0966608 -0.0389608 -0.0365888]  CS1Rot=[0.499609 0.399458 -0.768651;-0.217696 0.916751 0.334926;0.838451 0 0.544978]  CS2Pos=[0.0976595 -0.0366689 -0.0365888]  CS2Rot=[1 0 0;0 1 0;0 0 1]  CS3Pos=[0.0982587 -0.0352938 -0.0365888]  CS3Rot=[1 0 0;0 1 0;0 0 1]  CS4Pos=[0 0 0]  CS4Rot=[1 0 0;0 1 0;0 0 1]  CS5Pos=[]  CS5Rot=[]  CS6Pos=[]  CS6Rot=[]  CS7Pos=[]  CS7Rot=[]  CS8Pos=[]  CS8Rot=[]  CS9Pos=[]  CS9Rot=[]  CS10Pos=[]  CS10Rot=[]  CS11Pos=[]  CS11Rot=[]  CS12Pos=[]  CS12Rot=[]  CS13Pos=[]  CS13Rot=[]  CS14Pos=[]  CS14Rot=[]  CS15Pos=[]  CS15Rot=[]  CS16Pos=[]  CS16Rot=[]  CS17Pos=[]  CS17Rot=[]  CS18Pos=[]  CS18Rot=[]  CS19Pos=[]  CS19Rot=[]  CS20Pos=[]  CS20Rot=[]
  digit 5-2 : mblibv1/Bodies/Body  DialogController=MECH.DynMechDlgSource  PhysicalDomain=mechanical  SubClassName=Unknown  LeftPortType=workingframe  RightPortType=workingframe  LConnTagsString=CS2  RConnTagsString=CS3|CS4  UpdateFromCAD=on  DialogClass=MechanicalBodyBlock  Mass=0.000627913  MassUnits=kg  InertiaUnits=kg*m^2  Inertia=[4.77978e-009,7.52312e-009,6.57727e-010;7.52312e-009,4.69347e-007,-6.68752e-011;6.57727e-010,-6.68752e-011,4.65325e-007]  Shape=Cylinder  ShapeDims=[1 1]  ShapeUnits=m  ShapeUse=false  Density=1  DensityUnits=kg/m^3  DensityUse=false  GraphicsMode=GFXFILE  GraphicsFileName=Batbot - digit 5-2.STL  BodyColorSelMode=COLORPALETTE  BodyColor=[0.25098 0.25098 0.25098]  AttachedToCS=CS1  CG=Right$CG$[-0.130973 -0.0300504 -0.00748313]$WORLD$WORLD$m$[-0.229289 -0.343768 -0.910632;-0.0839379 0.939054 -0.333363;0.969732 0 -0.24417]$3x3 Transform$rad$WORLD$false$none  WorkingFrames=Right$CS1$[-0.126605 -0.0314785 -0.0226197]$WORLD$WORLD$m$[-0.229289 -0.343768 -0.910632;-0.0839379 0.939054 -0.333363;0.969732 0 -0.24417]$3x3 Transform$rad$WORLD$false$none#Left$CS2$[-0.12798 -0.0277222 -0.0226197]$WORLD$WORLD$m$[1 0 0;0 1 0;0 0 1]$3x3 Transform$rad$WORLD$true$none#Right$CS3$[-0.127464 -0.0291308 -0.0226197]$WORLD$WORLD$m$[1 0 0;0 1 0;0 0 1]$3x3 Transform$rad$WORLD$true$none#Right$CS4$[0 0 0]$WORLD$WORLD$m$[1 0 0;0 1 0;0 0 1]$3x3 Transform$rad$WORLD$true$none  CGPos=[-0.130973 -0.0300504 -0.00748313]  CGRot=[-0.229289 -0.343768 -0.910632;-0.0839379 0.939054 -0.333363;0.969732 0 -0.24417]  CS0Pos=[]  CS0Rot=[]  CS1Pos=[-0.126605 -0.0314785 -0.0226197]  CS1Rot=[-0.229289 -0.343768 -0.910632;-0.0839379 0.939054 -0.333363;0.969732 0 -0.24417]  CS2Pos=[-0.12798 -0.0277222 -0.0226197]  CS2Rot=[1 0 0;0 1 0;0 0 1]  CS3Pos=[-0.127464 -0.0291308 -0.0226197]  CS3Rot=[1 0 0;0 1 0;0 0 1]  CS4Pos=[0 0 0]  CS4Rot=[1 0 0;0 1 0;0 0 1]  CS5Pos=[]  CS5Rot=[]  CS6Pos=[]  CS6Rot=[]  CS7Pos=[]  CS7Rot=[]  CS8Pos=[]  CS8Rot=[]  CS9Pos=[]  CS9Rot=[]  CS10Pos=[]  CS10Rot=[]  CS11Pos=[]  CS11Rot=[]  CS12Pos=[]  CS12Rot=[]  CS13Pos=[]  CS13Rot=[]  CS14Pos=[]  CS14Rot=[]  CS15Pos=[]  CS15Rot=[]  CS16Pos=[]  CS16Rot=[]  CS17Pos=[]  CS17Rot=[]  CS18Pos=[]  CS18Rot=[]  CS19Pos=[]  CS19Rot=[]  CS20Pos=[]  CS20Rot=[]
  digit3-1 : mblibv1/Sensors &  Actuators/Body Sensor  DialogController=MECH.DynMechDlgSource  SystemSampleTime=-1  UpdateFromCAD=off  PhysicalDomain=Mechanical  PortType=blob  Muxed=off  Pose=on  Angle=on  AngleUnits=deg  ArcVelocity=off  ArcVelocityUnits=deg/s  ArcAcceleration=off  ArcAccelerationUnits=deg/s^2  CoordPosition=on  CoordPositionUnits=m  Velocity=off  VelocityUnits=m/s  Acceleration=off  AccelerationUnits=m/s^2  Quaternion=on  QuaternionDT=off  QuaternionDDT=off  QuaternionUnits=off  OutputVector=[1]  ActiveIO=on  Width=12  DialogClass=MechanicalSensorBlock  ReferenceFrame=Local (Body CS)
  digit3-2 : mblibv1/Sensors &  Actuators/Body Sensor  DialogController=MECH.DynMechDlgSource  SystemSampleTime=-1  UpdateFromCAD=off  PhysicalDomain=Mechanical  PortType=blob  Muxed=off  Pose=on  Angle=on  AngleUnits=deg  ArcVelocity=off  ArcVelocityUnits=deg/s  ArcAcceleration=off  ArcAccelerationUnits=deg/s^2  CoordPosition=on  CoordPositionUnits=m  Velocity=off  VelocityUnits=m/s  Acceleration=off  AccelerationUnits=m/s^2  Quaternion=on  QuaternionDT=off  QuaternionDDT=off  QuaternionUnits=off  OutputVector=[1]  ActiveIO=on  Width=12  DialogClass=MechanicalSensorBlock  ReferenceFrame=Local (Body CS)
  digit4-1 : mblibv1/Sensors &  Actuators/Body Sensor  DialogController=MECH.DynMechDlgSource  SystemSampleTime=-1  UpdateFromCAD=off  PhysicalDomain=Mechanical  PortType=blob  Muxed=off  Pose=on  Angle=on  AngleUnits=deg  ArcVelocity=off  ArcVelocityUnits=deg/s  ArcAcceleration=off  ArcAccelerationUnits=deg/s^2  CoordPosition=on  CoordPositionUnits=m  Velocity=off  VelocityUnits=m/s  Acceleration=off  AccelerationUnits=m/s^2  Quaternion=on  QuaternionDT=off  QuaternionDDT=off  QuaternionUnits=off  OutputVector=[1]  ActiveIO=on  Width=12  DialogClass=MechanicalSensorBlock  ReferenceFrame=Local (Body CS)
  digit4-2 : mblibv1/Sensors &  Actuators/Body Sensor  DialogController=MECH.DynMechDlgSource  SystemSampleTime=-1  UpdateFromCAD=off  PhysicalDomain=Mechanical  PortType=blob  Muxed=off  Pose=on  Angle=on  AngleUnits=deg  ArcVelocity=off  ArcVelocityUnits=deg/s  ArcAcceleration=off  ArcAccelerationUnits=deg/s^2  CoordPosition=on  CoordPositionUnits=m  Velocity=off  VelocityUnits=m/s  Acceleration=off  AccelerationUnits=m/s^2  Quaternion=on  QuaternionDT=off  QuaternionDDT=off  QuaternionUnits=off  OutputVector=[1]  ActiveIO=on  Width=12  DialogClass=MechanicalSensorBlock  ReferenceFrame=Local (Body CS)
  digit5-1 : mblibv1/Sensors &  Actuators/Body Sensor  DialogController=MECH.DynMechDlgSource  SystemSampleTime=-1  UpdateFromCAD=off  PhysicalDomain=Mechanical  PortType=blob  Muxed=off  Pose=on  Angle=on  AngleUnits=deg  ArcVelocity=off  ArcVelocityUnits=deg/s  ArcAcceleration=off  ArcAccelerationUnits=deg/s^2  CoordPosition=on  CoordPositionUnits=m  Velocity=off  VelocityUnits=m/s  Acceleration=off  AccelerationUnits=m/s^2  Quaternion=on  QuaternionDT=off  QuaternionDDT=off  QuaternionUnits=off  OutputVector=[1]  ActiveIO=on  Width=12  DialogClass=MechanicalSensorBlock  ReferenceFrame=Local (Body CS)
  digit5-2 : mblibv1/Sensors &  Actuators/Body Sensor  DialogController=MECH.DynMechDlgSource  SystemSampleTime=-1  UpdateFromCAD=off  PhysicalDomain=Mechanical  PortType=blob  Muxed=off  Pose=on  Angle=on  AngleUnits=deg  ArcVelocity=off  ArcVelocityUnits=deg/s  ArcAcceleration=off  ArcAccelerationUnits=deg/s^2  CoordPosition=on  CoordPositionUnits=m  Velocity=off  VelocityUnits=m/s  Acceleration=off  AccelerationUnits=m/s^2  Quaternion=on  QuaternionDT=off  QuaternionDDT=off  QuaternionUnits=off  OutputVector=[1]  ActiveIO=on  Width=12  DialogClass=MechanicalSensorBlock  ReferenceFrame=Local (Body CS)
  humerus-left : mblibv1/Sensors &  Actuators/Body Sensor  DialogController=MECH.DynMechDlgSource  SystemSampleTime=-1  UpdateFromCAD=off  PhysicalDomain=Mechanical  PortType=blob  Muxed=off  Pose=on  Angle=on  AngleUnits=deg  ArcVelocity=off  ArcVelocityUnits=deg/s  ArcAcceleration=off  ArcAccelerationUnits=deg/s^2  CoordPosition=on  CoordPositionUnits=m  Velocity=off  VelocityUnits=m/s  Acceleration=off  AccelerationUnits=m/s^2  Quaternion=on  QuaternionDT=off  QuaternionDDT=off  QuaternionUnits=off  OutputVector=[1]  ActiveIO=on  Width=12  DialogClass=MechanicalSensorBlock  ReferenceFrame=Local (Body CS)
  humerus-right : mblibv1/Sensors &  Actuators/Body Sensor  DialogController=MECH.DynMechDlgSource  SystemSampleTime=-1  UpdateFromCAD=off  PhysicalDomain=Mechanical  PortType=blob  Muxed=off  Pose=on  Angle=on  AngleUnits=deg  ArcVelocity=off  ArcVelocityUnits=deg/s  ArcAcceleration=off  ArcAccelerationUnits=deg/s^2  CoordPosition=on  CoordPositionUnits=m  Velocity=off  VelocityUnits=m/s  Acceleration=off  AccelerationUnits=m/s^2  Quaternion=on  QuaternionDT=off  QuaternionDDT=off  QuaternionUnits=off  OutputVector=[1]  ActiveIO=on  Width=12  DialogClass=MechanicalSensorBlock  ReferenceFrame=Local (Body CS)
  humerus5_left-1 : mblibv1/Bodies/Body  DialogController=MECH.DynMechDlgSource  PhysicalDomain=mechanical  SubClassName=Unknown  LeftPortType=workingframe  RightPortType=workingframe  LConnTagsString=CS2  RConnTagsString=CS3|CS4  UpdateFromCAD=on  DialogClass=MechanicalBodyBlock  Mass=0.00388478  MassUnits=kg  InertiaUnits=kg*m^2  Inertia=[9.8086e-008,-5.68803e-008,-2.88275e-009;-5.68803e-008,1.65963e-006,1.30066e-010;-2.88275e-009,1.30066e-010,1.71688e-006]  Shape=Cylinder  ShapeDims=[1 1]  ShapeUnits=m  ShapeUse=false  Density=1  DensityUnits=kg/m^3  DensityUse=false  GraphicsMode=GFXFILE  GraphicsFileName=Batbot - humerus5_left-1.STL  BodyColorSelMode=COLORPALETTE  BodyColor=[0.25098 0.25098 0.25098]  AttachedToCS=CS1  CG=Right$CG$[-0.0529655 -0.00265714 0.0100031]$WORLD$WORLD$m$[-0.766313 -0.542759 0.343768;-0.280531 -0.198693 -0.939054;0.577984 -0.816048 0]$3x3 Transform$rad$WORLD$false$none  WorkingFrames=Right$CS1$[-0.0389412 0.00284954 0]$WORLD$WORLD$m$[-0.766313 -0.542759 0.343768;-0.280531 -0.198693 -0.939054;0.577984 -0.816048 0]$3x3 Transform$rad$WORLD$false$none#Left$CS2$[-0.0401444 0.00613623 0]$WORLD$WORLD$m$[1 0 0;0 1 0;0 0 1]$3x3 Transform$rad$WORLD$true$none#Right$CS3$[-0.0841676 -0.0116836 0.0296556]$WORLD$WORLD$m$[1 0 0;0 1 0;0 0 1]$3x3 Transform$rad$WORLD$true$none#Right$CS4$[0 0 0]$WORLD$WORLD$m$[1 0 0;0 1 0;0 0 1]$3x3 Transform$rad$WORLD$true$none  CGPos=[-0.0529655 -0.00265714 0.0100031]  CGRot=[-0.766313 -0.542759 0.343768;-0.280531 -0.198693 -0.939054;0.577984 -0.816048 0]  CS0Pos=[]  CS0Rot=[]  CS1Pos=[-0.0389412 0.00284954 0]  CS1Rot=[-0.766313 -0.542759 0.343768;-0.280531 -0.198693 -0.939054;0.577984 -0.816048 0]  CS2Pos=[-0.0401444 0.00613623 0]  CS2Rot=[1 0 0;0 1 0;0 0 1]  CS3Pos=[-0.0841676 -0.0116836 0.0296556]  CS3Rot=[1 0 0;0 1 0;0 0 1]  CS4Pos=[0 0 0]  CS4Rot=[1 0 0;0 1 0;0 0 1]  CS5Pos=[]  CS5Rot=[]  CS6Pos=[]  CS6Rot=[]  CS7Pos=[]  CS7Rot=[]  CS8Pos=[]  CS8Rot=[]  CS9Pos=[]  CS9Rot=[]  CS10Pos=[]  CS10Rot=[]  CS11Pos=[]  CS11Rot=[]  CS12Pos=[]  CS12Rot=[]  CS13Pos=[]  CS13Rot=[]  CS14Pos=[]  CS14Rot=[]  CS15Pos=[]  CS15Rot=[]  CS16Pos=[]  CS16Rot=[]  CS17Pos=[]  CS17Rot=[]  CS18Pos=[]  CS18Rot=[]  CS19Pos=[]  CS19Rot=[]  CS20Pos=[]  CS20Rot=[]
  humerus5_right-1 : mblibv1/Bodies/Body  DialogController=MECH.DynMechDlgSource  PhysicalDomain=mechanical  SubClassName=Unknown  LeftPortType=workingframe  RightPortType=workingframe  LConnTagsString=CS2  RConnTagsString=CS3|CS4  UpdateFromCAD=on  DialogClass=MechanicalBodyBlock  Mass=0.0038586  MassUnits=kg  InertiaUnits=kg*m^2  Inertia=[9.77601e-008,-3.6228e-008,9.94906e-009;-3.6228e-008,1.68368e-006,-1.75654e-010;9.94906e-009,-1.75654e-010,1.73993e-006]  Shape=Cylinder  ShapeDims=[1 1]  ShapeUnits=m  ShapeUse=false  Density=1  DensityUnits=kg/m^3  DensityUse=false  GraphicsMode=GFXFILE  GraphicsFileName=Batbot - humerus5_right-1.STL  BodyColorSelMode=COLORPALETTE  BodyColor=[0.25098 0.25098 0.25098]  AttachedToCS=CS1  CG=Right$CG$[0.028644 -0.00412775 0.00731592]$WORLD$WORLD$m$[0.833143 0.3825 0.399458;-0.363027 -0.166668 0.916751;0.417234 -0.908799 0]$3x3 Transform$rad$WORLD$false$none  WorkingFrames=Right$CS1$[0.013305 0.00237779 -2.18943e-014]$WORLD$WORLD$m$[0.833143 0.3825 0.399458;-0.363027 -0.166668 0.916751;0.417234 -0.908799 0]$3x3 Transform$rad$WORLD$false$none#Left$CS2$[0.0149028 0.00604479 -2.18717e-014]$WORLD$WORLD$m$[1 0 0;0 1 0;0 0 1]$3x3 Transform$rad$WORLD$true$none#Right$CS3$[0.061853 -0.0167036 0.0203737]$WORLD$WORLD$m$[1 0 0;0 1 0;0 0 1]$3x3 Transform$rad$WORLD$true$none#Right$CS4$[0 0 0]$WORLD$WORLD$m$[1 0 0;0 1 0;0 0 1]$3x3 Transform$rad$WORLD$true$none  CGPos=[0.028644 -0.00412775 0.00731592]  CGRot=[0.833143 0.3825 0.399458;-0.363027 -0.166668 0.916751;0.417234 -0.908799 0]  CS0Pos=[]  CS0Rot=[]  CS1Pos=[0.013305 0.00237779 -2.18943e-014]  CS1Rot=[0.833143 0.3825 0.399458;-0.363027 -0.166668 0.916751;0.417234 -0.908799 0]  CS2Pos=[0.0149028 0.00604479 -2.18717e-014]  CS2Rot=[1 0 0;0 1 0;0 0 1]  CS3Pos=[0.061853 -0.0167036 0.0203737]  CS3Rot=[1 0 0;0 1 0;0 0 1]  CS4Pos=[0 0 0]  CS4Rot=[1 0 0;0 1 0;0 0 1]  CS5Pos=[]  CS5Rot=[]  CS6Pos=[]  CS6Rot=[]  CS7Pos=[]  CS7Rot=[]  CS8Pos=[]  CS8Rot=[]  CS9Pos=[]  CS9Rot=[]  CS10Pos=[]  CS10Rot=[]  CS11Pos=[]  CS11Rot=[]  CS12Pos=[]  CS12Rot=[]  CS13Pos=[]  CS13Rot=[]  CS14Pos=[]  CS14Rot=[]  CS15Pos=[]  CS15Rot=[]  CS16Pos=[]  CS16Rot=[]  CS17Pos=[]  CS17Rot=[]  CS18Pos=[]  CS18Rot=[]  CS19Pos=[]  CS19Rot=[]  CS20Pos=[]  CS20Rot=[]
  leg-1 : mblibv1/Bodies/Body  DialogController=MECH.DynMechDlgSource  PhysicalDomain=mechanical  SubClassName=Unknown  LeftPortType=workingframe  RightPortType=workingframe  LConnTagsString=CS2  UpdateFromCAD=on  DialogClass=MechanicalBodyBlock  Mass=0.000873585  MassUnits=kg  InertiaUnits=kg*m^2  Inertia=[6.16178e-008,1.7833e-015,-7.80759e-008;1.7833e-015,1.78974e-007,-9.84923e-016;-7.80759e-008,-9.84923e-016,1.19394e-007]  Shape=Cylinder  ShapeDims=[1 1]  ShapeUnits=m  ShapeUse=false  Density=1  DensityUnits=kg/m^3  DensityUse=false  GraphicsMode=GFXFILE  GraphicsFileName=Batbot - leg-1.STL  BodyColorSelMode=COLORPALETTE  BodyColor=[0.25098;0.25098;0.25098]  AttachedToCS=CS1  CG=Right$CG$[0.0220297 0.00238611 0.066232]$WORLD$WORLD$m$[0.894466 0 -0.447136;0 1 0;0.447136 0 0.894466]$3x3 Transform$rad$WORLD$false$none  WorkingFrames=Right$CS1$[0.0112651 0.00038611 0.052]$WORLD$WORLD$m$[0.894466 0 -0.447136;0 1 0;0.447136 0 0.894466]$3x3 Transform$rad$WORLD$false$none#Left$CS2$[0.0112651 0.00438611 0.052]$WORLD$WORLD$m$[1 0 0;0 1 0;0 0 1]$3x3 Transform$rad$WORLD$true$none  CGPos=[0.0220297 0.00238611 0.066232]  CGRot=[0.894466 0 -0.447136;0 1 0;0.447136 0 0.894466]  CS0Pos=[]  CS0Rot=[]  CS1Pos=[0.0112651 0.00038611 0.052]  CS1Rot=[0.894466 0 -0.447136;0 1 0;0.447136 0 0.894466]  CS2Pos=[0.0112651 0.00438611 0.052]  CS2Rot=[1 0 0;0 1 0;0 0 1]  CS3Pos=[]  CS3Rot=[]  CS4Pos=[]  CS4Rot=[]  CS5Pos=[]  CS5Rot=[]  CS6Pos=[]  CS6Rot=[]  CS7Pos=[]  CS7Rot=[]  CS8Pos=[]  CS8Rot=[]  CS9Pos=[]  CS9Rot=[]  CS10Pos=[]  CS10Rot=[]  CS11Pos=[]  CS11Rot=[]  CS12Pos=[]  CS12Rot=[]  CS13Pos=[]  CS13Rot=[]  CS14Pos=[]  CS14Rot=[]  CS15Pos=[]  CS15Rot=[]  CS16Pos=[]  CS16Rot=[]  CS17Pos=[]  CS17Rot=[]  CS18Pos=[]  CS18Rot=[]  CS19Pos=[]  CS19Rot=[]  CS20Pos=[]  CS20Rot=[]
  leg-2 : mblibv1/Bodies/Body  DialogController=MECH.DynMechDlgSource  PhysicalDomain=mechanical  SubClassName=Unknown  LeftPortType=workingframe  RightPortType=workingframe  LConnTagsString=CS2  UpdateFromCAD=on  DialogClass=MechanicalBodyBlock  Mass=0.000873585  MassUnits=kg  InertiaUnits=kg*m^2  Inertia=[6.16178e-008,1.7833e-015,-7.80759e-008;1.7833e-015,1.78974e-007,-9.84923e-016;-7.80759e-008,-9.84923e-016,1.19394e-007]  Shape=Cylinder  ShapeDims=[1 1]  ShapeUnits=m  ShapeUse=false  Density=1  DensityUnits=kg/m^3  DensityUse=false  GraphicsMode=GFXFILE  GraphicsFileName=Batbot - leg-2.STL  BodyColorSelMode=COLORPALETTE  BodyColor=[0.25098;0.25098;0.25098]  AttachedToCS=CS1  CG=Right$CG$[-0.0442793 0.00238611 0.0681713]$WORLD$WORLD$m$[-0.780947 0 0.624598;0 -1 0;0.624598 0 0.780947]$3x3 Transform$rad$WORLD$false$none  WorkingFrames=Right$CS1$[-0.0367349 0.00438611 0.052]$WORLD$WORLD$m$[-0.780947 0 0.624598;0 -1 0;0.624598 0 0.780947]$3x3 Transform$rad$WORLD$false$none#Left$CS2$[-0.0367349 0.00438611 0.052]$WORLD$WORLD$m$[1 0 0;0 1 0;0 0 1]$3x3 Transform$rad$WORLD$true$none  CGPos=[-0.0442793 0.00238611 0.0681713]  CGRot=[-0.780947 0 0.624598;0 -1 0;0.624598 0 0.780947]  CS0Pos=[]  CS0Rot=[]  CS1Pos=[-0.0367349 0.00438611 0.052]  CS1Rot=[-0.780947 0 0.624598;0 -1 0;0.624598 0 0.780947]  CS2Pos=[-0.0367349 0.00438611 0.052]  CS2Rot=[1 0 0;0 1 0;0 0 1]  CS3Pos=[]  CS3Rot=[]  CS4Pos=[]  CS4Rot=[]  CS5Pos=[]  CS5Rot=[]  CS6Pos=[]  CS6Rot=[]  CS7Pos=[]  CS7Rot=[]  CS8Pos=[]  CS8Rot=[]  CS9Pos=[]  CS9Rot=[]  CS10Pos=[]  CS10Rot=[]  CS11Pos=[]  CS11Rot=[]  CS12Pos=[]  CS12Rot=[]  CS13Pos=[]  CS13Rot=[]  CS14Pos=[]  CS14Rot=[]  CS15Pos=[]  CS15Rot=[]  CS16Pos=[]  CS16Rot=[]  CS17Pos=[]  CS17Rot=[]  CS18Pos=[]  CS18Rot=[]  CS19Pos=[]  CS19Rot=[]  CS20Pos=[]  CS20Rot=[]
  motor_case-2 : mblibv1/Bodies/Body  DialogController=MECH.DynMechDlgSource  PhysicalDomain=mechanical  SubClassName=Unknown  LeftPortType=workingframe  RightPortType=workingframe  LConnTagsString=CS3|CS4  RConnTagsString=CS2  UpdateFromCAD=on  DialogClass=MechanicalBodyBlock  Mass=0.00589266  MassUnits=kg  InertiaUnits=kg*m^2  Inertia=[1.45703e-006,6.98041e-010,2.27921e-011;6.98041e-010,2.88185e-007,6.12252e-009;2.27921e-011,6.12252e-009,1.49863e-006]  Shape=Cylinder  ShapeDims=[1 1]  ShapeUnits=m  ShapeUse=false  Density=1  DensityUnits=kg/m^3  DensityUse=false  GraphicsMode=GFXFILE  GraphicsFileName=Batbot - motor_case-2.STL  BodyColorSelMode=COLORPALETTE  BodyColor=[0.25098;0.25098;0.25098]  AttachedToCS=CS1  CG=Right$CG$[-0.0127433 0.00186569 0.0266734]$WORLD$WORLD$m$[1 0 0;0 1 0;0 0 1]$3x3 Transform$rad$WORLD$false$none  WorkingFrames=Right$CS1$[0.00126505 0.00078611 -2.18437e-014]$WORLD$WORLD$m$[1 0 0;0 1 0;0 0 1]$3x3 Transform$rad$WORLD$false$none#Right$CS2$[-0.0189849 0.0235361 0.0355]$WORLD$WORLD$m$[1 0 0;0 1 0;0 0 1]$3x3 Transform$rad$WORLD$true$none#Left$CS3$[-0.00498495 -0.0167139 0.019]$WORLD$WORLD$m$[1 0 0;0 1 0;0 0 1]$3x3 Transform$rad$WORLD$true$none#Left$CS4$[-0.00498495 -0.0167139 0.019]$WORLD$WORLD$m$[1 0 0;0 1 0;0 0 1]$3x3 Transform$rad$WORLD$true$none  CGPos=[-0.0127433 0.00186569 0.0266734]  CGRot=[1 0 0;0 1 0;0 0 1]  CS0Pos=[]  CS0Rot=[]  CS1Pos=[0.00126505 0.00078611 -2.18437e-014]  CS1Rot=[1 0 0;0 1 0;0 0 1]  CS2Pos=[-0.0189849 0.0235361 0.0355]  CS2Rot=[1 0 0;0 1 0;0 0 1]  CS3Pos=[-0.00498495 -0.0167139 0.019]  CS3Rot=[1 0 0;0 1 0;0 0 1]  CS4Pos=[-0.00498495 -0.0167139 0.019]  CS4Rot=[1 0 0;0 1 0;0 0 1]  CS5Pos=[]  CS5Rot=[]  CS6Pos=[]  CS6Rot=[]  CS7Pos=[]  CS7Rot=[]  CS8Pos=[]  CS8Rot=[]  CS9Pos=[]  CS9Rot=[]  CS10Pos=[]  CS10Rot=[]  CS11Pos=[]  CS11Rot=[]  CS12Pos=[]  CS12Rot=[]  CS13Pos=[]  CS13Rot=[]  CS14Pos=[]  CS14Rot=[]  CS15Pos=[]  CS15Rot=[]  CS16Pos=[]  CS16Rot=[]  CS17Pos=[]  CS17Rot=[]  CS18Pos=[]  CS18Rot=[]  CS19Pos=[]  CS19Rot=[]  CS20Pos=[]  CS20Rot=[]
  radius-left : mblibv1/Sensors &  Actuators/Body Sensor  DialogController=MECH.DynMechDlgSource  SystemSampleTime=-1  UpdateFromCAD=off  PhysicalDomain=Mechanical  PortType=blob  Muxed=off  Pose=on  Angle=on  AngleUnits=deg  ArcVelocity=off  ArcVelocityUnits=deg/s  ArcAcceleration=off  ArcAccelerationUnits=deg/s^2  CoordPosition=on  CoordPositionUnits=m  Velocity=off  VelocityUnits=m/s  Acceleration=off  AccelerationUnits=m/s^2  Quaternion=on  QuaternionDT=off  QuaternionDDT=off  QuaternionUnits=off  OutputVector=[1]  ActiveIO=on  Width=12  DialogClass=MechanicalSensorBlock  ReferenceFrame=Local (Body CS)
  radius-right : mblibv1/Sensors &  Actuators/Body Sensor  DialogController=MECH.DynMechDlgSource  SystemSampleTime=-1  UpdateFromCAD=off  PhysicalDomain=Mechanical  PortType=blob  Muxed=off  Pose=on  Angle=on  AngleUnits=deg  ArcVelocity=off  ArcVelocityUnits=deg/s  ArcAcceleration=off  ArcAccelerationUnits=deg/s^2  CoordPosition=on  CoordPositionUnits=m  Velocity=off  VelocityUnits=m/s  Acceleration=off  AccelerationUnits=m/s^2  Quaternion=on  QuaternionDT=off  QuaternionDDT=off  QuaternionUnits=off  OutputVector=[1]  ActiveIO=on  Width=12  DialogClass=MechanicalSensorBlock  ReferenceFrame=Local (Body CS)
  radius5-1 : mblibv1/Bodies/Body  DialogController=MECH.DynMechDlgSource  PhysicalDomain=mechanical  SubClassName=Unknown  LeftPortType=workingframe  RightPortType=workingframe  LConnTagsString=CS2  RConnTagsString=CS3|CS4|CS5  UpdateFromCAD=on  DialogClass=MechanicalBodyBlock  Mass=0.00250557  MassUnits=kg  InertiaUnits=kg*m^2  Inertia=[3.6957e-008,-1.71957e-008,-5.01752e-008;-1.71957e-008,1.75521e-006,-7.17954e-010;-5.01752e-008,-7.17954e-010,1.74444e-006]  Shape=Cylinder  ShapeDims=[1 1]  ShapeUnits=m  ShapeUse=false  Density=1  DensityUnits=kg/m^3  DensityUse=false  GraphicsMode=GFXFILE  GraphicsFileName=Batbot - radius5-1.STL  BodyColorSelMode=COLORPALETTE  BodyColor=[0.25098 0.25098 0.25098]  AttachedToCS=CS1  CG=Right$CG$[0.0831116 -0.0274789 -0.0115511]$WORLD$WORLD$m$[0.500637 0.399458 0.767982;-0.218144 0.916751 -0.334634;-0.837721 0 0.546099]$3x3 Transform$rad$WORLD$false$none  WorkingFrames=Right$CS1$[0.0619599 -0.0227496 0.022012]$WORLD$WORLD$m$[0.500637 0.399458 0.767982;-0.218144 0.916751 -0.334634;-0.837721 0 0.546099]$3x3 Transform$rad$WORLD$false$none#Left$CS2$[0.061853 -0.0167036 0.0203737]$WORLD$WORLD$m$[1 0 0;0 1 0;0 0 1]$3x3 Transform$rad$WORLD$true$none#Right$CS3$[0.0976595 -0.0366689 -0.0365888]$WORLD$WORLD$m$[1 0 0;0 1 0;0 0 1]$3x3 Transform$rad$WORLD$true$none#Right$CS4$[0.0996967 -0.0319935 -0.0365888]$WORLD$WORLD$m$[1 0 0;0 1 0;0 0 1]$3x3 Transform$rad$WORLD$true$none#Right$CS5$[0 0 0]$WORLD$WORLD$m$[1 0 0;0 1 0;0 0 1]$3x3 Transform$rad$WORLD$true$none  CGPos=[0.0831116 -0.0274789 -0.0115511]  CGRot=[0.500637 0.399458 0.767982;-0.218144 0.916751 -0.334634;-0.837721 0 0.546099]  CS0Pos=[]  CS0Rot=[]  CS1Pos=[0.0619599 -0.0227496 0.022012]  CS1Rot=[0.500637 0.399458 0.767982;-0.218144 0.916751 -0.334634;-0.837721 0 0.546099]  CS2Pos=[0.061853 -0.0167036 0.0203737]  CS2Rot=[1 0 0;0 1 0;0 0 1]  CS3Pos=[0.0976595 -0.0366689 -0.0365888]  CS3Rot=[1 0 0;0 1 0;0 0 1]  CS4Pos=[0.0996967 -0.0319935 -0.0365888]  CS4Rot=[1 0 0;0 1 0;0 0 1]  CS5Pos=[0 0 0]  CS5Rot=[1 0 0;0 1 0;0 0 1]  CS6Pos=[]  CS6Rot=[]  CS7Pos=[]  CS7Rot=[]  CS8Pos=[]  CS8Rot=[]  CS9Pos=[]  CS9Rot=[]  CS10Pos=[]  CS10Rot=[]  CS11Pos=[]  CS11Rot=[]  CS12Pos=[]  CS12Rot=[]  CS13Pos=[]  CS13Rot=[]  CS14Pos=[]  CS14Rot=[]  CS15Pos=[]  CS15Rot=[]  CS16Pos=[]  CS16Rot=[]  CS17Pos=[]  CS17Rot=[]  CS18Pos=[]  CS18Rot=[]  CS19Pos=[]  CS19Rot=[]  CS20Pos=[]  CS20Rot=[]
  radius5-2 : mblibv1/Bodies/Body  DialogController=MECH.DynMechDlgSource  PhysicalDomain=mechanical  SubClassName=Unknown  LeftPortType=workingframe  RightPortType=workingframe  LConnTagsString=CS2  RConnTagsString=CS3|CS4|CS5  UpdateFromCAD=on  DialogClass=MechanicalBodyBlock  Mass=0.00250557  MassUnits=kg  InertiaUnits=kg*m^2  Inertia=[3.6957e-008,-1.71957e-008,-5.01752e-008;-1.71957e-008,1.75521e-006,-7.17954e-010;-5.01752e-008,-7.17954e-010,1.74444e-006]  Shape=Cylinder  ShapeDims=[1 1]  ShapeUnits=m  ShapeUse=false  Density=1  DensityUnits=kg/m^3  DensityUse=false  GraphicsMode=GFXFILE  GraphicsFileName=Batbot - radius5-2.STL  BodyColorSelMode=COLORPALETTE  BodyColor=[0.25098 0.25098 0.25098]  AttachedToCS=CS1  CG=Right$CG$[-0.108688 -0.0234434 0.000456752]$WORLD$WORLD$m$[-0.593958 0.343768 -0.727349;-0.217436 -0.939054 -0.266267;-0.774555 0 0.632507]$3x3 Transform$rad$WORLD$false$none  WorkingFrames=Right$CS1$[-0.0868653 -0.0110738 0.0315531]$WORLD$WORLD$m$[-0.593958 0.343768 -0.727349;-0.217436 -0.939054 -0.266267;-0.774555 0 0.632507]$3x3 Transform$rad$WORLD$false$none#Left$CS2$[-0.0841676 -0.0116836 0.0296556]$WORLD$WORLD$m$[1 0 0;0 1 0;0 0 1]$3x3 Transform$rad$WORLD$true$none#Right$CS3$[-0.12798 -0.0277222 -0.0226197]$WORLD$WORLD$m$[1 0 0;0 1 0;0 0 1]$3x3 Transform$rad$WORLD$true$none#Right$CS4$[-0.126226 -0.0325114 -0.0226197]$WORLD$WORLD$m$[1 0 0;0 1 0;0 0 1]$3x3 Transform$rad$WORLD$true$none#Right$CS5$[0 0 0]$WORLD$WORLD$m$[1 0 0;0 1 0;0 0 1]$3x3 Transform$rad$WORLD$true$none  CGPos=[-0.108688 -0.0234434 0.000456752]  CGRot=[-0.593958 0.343768 -0.727349;-0.217436 -0.939054 -0.266267;-0.774555 0 0.632507]  CS0Pos=[]  CS0Rot=[]  CS1Pos=[-0.0868653 -0.0110738 0.0315531]  CS1Rot=[-0.593958 0.343768 -0.727349;-0.217436 -0.939054 -0.266267;-0.774555 0 0.632507]  CS2Pos=[-0.0841676 -0.0116836 0.0296556]  CS2Rot=[1 0 0;0 1 0;0 0 1]  CS3Pos=[-0.12798 -0.0277222 -0.0226197]  CS3Rot=[1 0 0;0 1 0;0 0 1]  CS4Pos=[-0.126226 -0.0325114 -0.0226197]  CS4Rot=[1 0 0;0 1 0;0 0 1]  CS5Pos=[0 0 0]  CS5Rot=[1 0 0;0 1 0;0 0 1]  CS6Pos=[]  CS6Rot=[]  CS7Pos=[]  CS7Rot=[]  CS8Pos=[]  CS8Rot=[]  CS9Pos=[]  CS9Rot=[]  CS10Pos=[]  CS10Rot=[]  CS11Pos=[]  CS11Rot=[]  CS12Pos=[]  CS12Rot=[]  CS13Pos=[]  CS13Rot=[]  CS14Pos=[]  CS14Rot=[]  CS15Pos=[]  CS15Rot=[]  CS16Pos=[]  CS16Rot=[]  CS17Pos=[]  CS17Rot=[]  CS18Pos=[]  CS18Rot=[]  CS19Pos=[]  CS19Rot=[]  CS20Pos=[]  CS20Rot=[]
  servo-1 : mblibv1/Bodies/Body  DialogController=MECH.DynMechDlgSource  PhysicalDomain=mechanical  SubClassName=Unknown  LeftPortType=workingframe  RightPortType=workingframe  LConnTagsString=CS3  RConnTagsString=CS2  UpdateFromCAD=on  DialogClass=MechanicalBodyBlock  Mass=0.00760085  MassUnits=kg  InertiaUnits=kg*m^2  Inertia=[6.91379e-007,3.2892e-012,9.73497e-012;3.2892e-012,4.21849e-007,-3.81458e-008;9.73497e-012,-3.81458e-008,4.47884e-007]  Shape=Cylinder  ShapeDims=[1 1]  ShapeUnits=m  ShapeUse=false  Density=1  DensityUnits=kg/m^3  DensityUse=false  GraphicsMode=GFXFILE  GraphicsFileName=Batbot - servo-1.STL  BodyColorSelMode=COLORPALETTE  BodyColor=[0;0;1]  AttachedToCS=CS1  CG=Right$CG$[-0.0124599 0.0124729 0.0225887]$WORLD$WORLD$m$[-1 0 0;0 1 0;0 0 -1]$3x3 Transform$rad$WORLD$false$none  WorkingFrames=Right$CS1$[-0.00645995 0.00053611 0.0135]$WORLD$WORLD$m$[-1 0 0;0 1 0;0 0 -1]$3x3 Transform$rad$WORLD$false$none#Right$CS2$[-0.0124493 0.017571 0.0095]$WORLD$WORLD$m$[1 0 0;0 1 0;0 0 1]$3x3 Transform$rad$WORLD$true$none#Left$CS3$[-0.0189849 0.0235361 0.0355]$WORLD$WORLD$m$[1 0 0;0 1 0;0 0 1]$3x3 Transform$rad$WORLD$true$none  CGPos=[-0.0124599 0.0124729 0.0225887]  CGRot=[-1 0 0;0 1 0;0 0 -1]  CS0Pos=[]  CS0Rot=[]  CS1Pos=[-0.00645995 0.00053611 0.0135]  CS1Rot=[-1 0 0;0 1 0;0 0 -1]  CS2Pos=[-0.0124493 0.017571 0.0095]  CS2Rot=[1 0 0;0 1 0;0 0 1]  CS3Pos=[-0.0189849 0.0235361 0.0355]  CS3Rot=[1 0 0;0 1 0;0 0 1]  CS4Pos=[]  CS4Rot=[]  CS5Pos=[]  CS5Rot=[]  CS6Pos=[]  CS6Rot=[]  CS7Pos=[]  CS7Rot=[]  CS8Pos=[]  CS8Rot=[]  CS9Pos=[]  CS9Rot=[]  CS10Pos=[]  CS10Rot=[]  CS11Pos=[]  CS11Rot=[]  CS12Pos=[]  CS12Rot=[]  CS13Pos=[]  CS13Rot=[]  CS14Pos=[]  CS14Rot=[]  CS15Pos=[]  CS15Rot=[]  CS16Pos=[]  CS16Rot=[]  CS17Pos=[]  CS17Rot=[]  CS18Pos=[]  CS18Rot=[]  CS19Pos=[]  CS19Rot=[]  CS20Pos=[]  CS20Rot=[]
  shoulder-left : mblibv1/Sensors &  Actuators/Body Sensor  DialogController=MECH.DynMechDlgSource  SystemSampleTime=-1  UpdateFromCAD=off  PhysicalDomain=Mechanical  PortType=blob  Muxed=off  Pose=on  Angle=on  AngleUnits=deg  ArcVelocity=off  ArcVelocityUnits=deg/s  ArcAcceleration=off  ArcAccelerationUnits=deg/s^2  CoordPosition=on  CoordPositionUnits=m  Velocity=off  VelocityUnits=m/s  Acceleration=off  AccelerationUnits=m/s^2  Quaternion=on  QuaternionDT=off  QuaternionDDT=off  QuaternionUnits=off  OutputVector=[1]  ActiveIO=on  Width=12  DialogClass=MechanicalSensorBlock  ReferenceFrame=Local (Body CS)
  shoulder-right : mblibv1/Sensors &  Actuators/Body Sensor  DialogController=MECH.DynMechDlgSource  SystemSampleTime=-1  UpdateFromCAD=off  PhysicalDomain=Mechanical  PortType=blob  Muxed=off  Pose=on  Angle=on  AngleUnits=deg  ArcVelocity=off  ArcVelocityUnits=deg/s  ArcAcceleration=off  ArcAccelerationUnits=deg/s^2  CoordPosition=on  CoordPositionUnits=m  Velocity=off  VelocityUnits=m/s  Acceleration=off  AccelerationUnits=m/s^2  Quaternion=on  QuaternionDT=off  QuaternionDDT=off  QuaternionUnits=off  OutputVector=[1]  ActiveIO=on  Width=12  DialogClass=MechanicalSensorBlock  ReferenceFrame=Local (Body CS)
  shoulder5_left-1 : mblibv1/Bodies/Body  DialogController=MECH.DynMechDlgSource  PhysicalDomain=mechanical  SubClassName=Unknown  LeftPortType=workingframe  RightPortType=workingframe  LConnTagsString=CS2  RConnTagsString=CS3|CS4|CS5  UpdateFromCAD=on  DialogClass=MechanicalBodyBlock  Mass=0.00901241  MassUnits=kg  InertiaUnits=kg*m^2  Inertia=[2.00808e-006,6.76412e-008,2.46891e-009;6.76412e-008,6.63601e-007,1.33885e-009;2.46891e-009,1.33885e-009,1.59987e-006]  Shape=Cylinder  ShapeDims=[1 1]  ShapeUnits=m  ShapeUse=false  Density=1  DensityUnits=kg/m^3  DensityUse=false  GraphicsMode=GFXFILE  GraphicsFileName=Batbot - shoulder5_left-1.STL  BodyColorSelMode=COLORPALETTE  BodyColor=[0.25098 0.25098 0.25098]  AttachedToCS=CS1  CG=Right$CG$[-0.0413208 0.00144688 0.00594565]$WORLD$WORLD$m$[-0.939054 0 -0.343768;-0.343768 0 0.939054;0 1 0]$3x3 Transform$rad$WORLD$false$none  WorkingFrames=Right$CS1$[-0.0387349 0.00228611 0]$WORLD$WORLD$m$[-0.939054 0 -0.343768;-0.343768 0 0.939054;0 1 0]$3x3 Transform$rad$WORLD$false$none#Left$CS2$[-0.0387349 0.00228611 0.034]$WORLD$WORLD$m$[1 0 0;0 1 0;0 0 1]$3x3 Transform$rad$WORLD$true$none#Right$CS3$[-0.0401444 0.00613623 0]$WORLD$WORLD$m$[1 0 0;0 1 0;0 0 1]$3x3 Transform$rad$WORLD$true$none#Right$CS4$[-0.0446993 0.0185787 0.005]$WORLD$WORLD$m$[1 0 0;0 1 0;0 0 1]$3x3 Transform$rad$WORLD$true$none#Right$CS5$[0 0 0]$WORLD$WORLD$m$[1 0 0;0 1 0;0 0 1]$3x3 Transform$rad$WORLD$true$none  CGPos=[-0.0413208 0.00144688 0.00594565]  CGRot=[-0.939054 0 -0.343768;-0.343768 0 0.939054;0 1 0]  CS0Pos=[]  CS0Rot=[]  CS1Pos=[-0.0387349 0.00228611 0]  CS1Rot=[-0.939054 0 -0.343768;-0.343768 0 0.939054;0 1 0]  CS2Pos=[-0.0387349 0.00228611 0.034]  CS2Rot=[1 0 0;0 1 0;0 0 1]  CS3Pos=[-0.0401444 0.00613623 0]  CS3Rot=[1 0 0;0 1 0;0 0 1]  CS4Pos=[-0.0446993 0.0185787 0.005]  CS4Rot=[1 0 0;0 1 0;0 0 1]  CS5Pos=[0 0 0]  CS5Rot=[1 0 0;0 1 0;0 0 1]  CS6Pos=[]  CS6Rot=[]  CS7Pos=[]  CS7Rot=[]  CS8Pos=[]  CS8Rot=[]  CS9Pos=[]  CS9Rot=[]  CS10Pos=[]  CS10Rot=[]  CS11Pos=[]  CS11Rot=[]  CS12Pos=[]  CS12Rot=[]  CS13Pos=[]  CS13Rot=[]  CS14Pos=[]  CS14Rot=[]  CS15Pos=[]  CS15Rot=[]  CS16Pos=[]  CS16Rot=[]  CS17Pos=[]  CS17Rot=[]  CS18Pos=[]  CS18Rot=[]  CS19Pos=[]  CS19Rot=[]  CS20Pos=[]  CS20Rot=[]
  shoulder5_right-1 : mblibv1/Bodies/Body  DialogController=MECH.DynMechDlgSource  PhysicalDomain=mechanical  SubClassName=Unknown  LeftPortType=workingframe  RightPortType=workingframe  LConnTagsString=CS3  RConnTagsString=CS2|CS4|CS5  UpdateFromCAD=on  DialogClass=MechanicalBodyBlock  Mass=0.00901257  MassUnits=kg  InertiaUnits=kg*m^2  Inertia=[2.00808e-006,6.76379e-008,-3.06892e-009;6.76379e-008,6.63619e-007,-2.62474e-009;-3.06892e-009,-2.62474e-009,1.59986e-006]  Shape=Cylinder  ShapeDims=[1 1]  ShapeUnits=m  ShapeUse=false  Density=1  DensityUnits=kg/m^3  DensityUse=false  GraphicsMode=GFXFILE  GraphicsFileName=Batbot - shoulder5_right-1.STL  BodyColorSelMode=COLORPALETTE  BodyColor=[0.25098 0.25098 0.25098]  AttachedToCS=CS1  CG=Right$CG$[0.0158057 0.00131584 0.00594558]$WORLD$WORLD$m$[0.916751 0 -0.399458;-0.399458 0 -0.916751;0 1 0]$3x3 Transform$rad$WORLD$false$none  WorkingFrames=Right$CS1$[0.0132651 0.00228611 -2.18454e-014]$WORLD$WORLD$m$[0.916751 0 -0.399458;-0.399458 0 -0.916751;0 1 0]$3x3 Transform$rad$WORLD$false$none#Right$CS2$[0.0201957 0.0181917 0.005]$WORLD$WORLD$m$[1 0 0;0 1 0;0 0 1]$3x3 Transform$rad$WORLD$true$none#Left$CS3$[0.0132651 0.00228611 0.034]$WORLD$WORLD$m$[1 0 0;0 1 0;0 0 1]$3x3 Transform$rad$WORLD$true$none#Right$CS4$[0.0149028 0.00604479 -2.18717e-014]$WORLD$WORLD$m$[1 0 0;0 1 0;0 0 1]$3x3 Transform$rad$WORLD$true$none#Right$CS5$[0 0 0]$World$World$m$[1 0 0;0 1 0;0 0 1]$3x3 Transform$rad$World$true$none  CGPos=[0.0158057 0.00131584 0.00594558]  CGRot=[0.916751 0 -0.399458;-0.399458 0 -0.916751;0 1 0]  CS0Pos=[]  CS0Rot=[]  CS1Pos=[0.0132651 0.00228611 -2.18454e-014]  CS1Rot=[0.916751 0 -0.399458;-0.399458 0 -0.916751;0 1 0]  CS2Pos=[0.0201957 0.0181917 0.005]  CS2Rot=[1 0 0;0 1 0;0 0 1]  CS3Pos=[0.0132651 0.00228611 0.034]  CS3Rot=[1 0 0;0 1 0;0 0 1]  CS4Pos=[0.0149028 0.00604479 -2.18717e-014]  CS4Rot=[1 0 0;0 1 0;0 0 1]  CS5Pos=[0 0 0]  CS5Rot=[1 0 0;0 1 0;0 0 1]  CS6Pos=[]  CS6Rot=[]  CS7Pos=[]  CS7Rot=[]  CS8Pos=[]  CS8Rot=[]  CS9Pos=[]  CS9Rot=[]  CS10Pos=[]  CS10Rot=[]  CS11Pos=[]  CS11Rot=[]  CS12Pos=[]  CS12Rot=[]  CS13Pos=[]  CS13Rot=[]  CS14Pos=[]  CS14Rot=[]  CS15Pos=[]  CS15Rot=[]  CS16Pos=[]  CS16Rot=[]  CS17Pos=[]  CS17Rot=[]  CS18Pos=[]  CS18Rot=[]  CS19Pos=[]  CS19Rot=[]  CS20Pos=[]  CS20Rot=[]
  Flapping_Angle : Outport  OutDataType=fixdt(1, 16)  OutScaling=2^0
  HumerusLEFT_Angle : Outport  Port=2  OutDataType=fixdt(1, 16)  OutScaling=2^0
  RadiusLEFT_Angle : Outport  Port=3  OutDataType=fixdt(1, 16)  OutScaling=2^0
  HumerusRIGHT_Angle : Outport  Port=4  OutDataType=fixdt(1, 16)  OutScaling=2^0
  RadiusRIGHT_Angle : Outport  Port=5  OutDataType=fixdt(1, 16)  OutScaling=2^0
  Base_POS : Outport  Port=6  OutDataType=fixdt(1, 16)  OutScaling=2^0
  Base_Angles : Outport  Port=7  OutDataType=fixdt(1, 16)  OutScaling=2^0
  tag scope: F_R=global, F_p=global, Flapping=global, HL_R=global, HL_p=global, HR_R=global, HR_p=global, Humerus_L=global, Humerus_R=global, RL_R=global, RL_p=global, RR_R=global, RR_p=global, Radius_L=global, Radius_R=global, SL_R=global, SL_p=global, SR_R=global, SR_p=global, d31_R=global, d31_p=global, d32_R=global, d32_p=global, d41_R=global, d41_p=global, d42_R=global, d42_p=global, d51_R=global, d51_p=global, d52_R=global, d52_p=global, fb_R=global, fb_p=global, legs=global, wrist_L=global, wrist_R=global
  wires:
  Floating-base/1 -> [fb_p]
  Floating-base/2 -> [fb_R]
  shoulder-right/1 -> [SR_p]
  shoulder-right/2 -> [SR_R]
  shoulder-left/1 -> [SL_p]
  shoulder-left/2 -> [SL_R]
  humerus-left/1 -> [HL_p]
  humerus-left/2 -> [HL_R]
  humerus-right/1 -> [HR_p]
  humerus-right/2 -> [HR_R]
  radius-right/1 -> [RR_p]
  radius-right/2 -> [RR_R]
  radius-left/1 -> [RL_p]
  radius-left/2 -> [RL_R]
  digit5-1/1 -> [d51_p]
  digit5-1/2 -> [d51_R]
  digit3-1/2 -> [d31_R]
  digit3-1/1 -> [d31_p]
  digit4-1/2 -> [d41_R]
  digit4-1/1 -> [d41_p]
  digit5-2/1 -> [d52_p]
  digit5-2/2 -> [d52_R]
  digit3-2/2 -> [d32_R]
  digit3-2/1 -> [d32_p]
  digit4-2/2 -> [d42_R]
  digit4-2/1 -> [d42_p]
  [Humerus_L] -> Joint Actuator2/1
  [Humerus_R] -> Joint Actuator1/1
  [Flapping] -> Joint Actuator/1
  [Radius_R] -> Joint Actuator4/1
  [Radius_L] -> Joint Actuator3/1
  [wrist_R] -> Gain1/1
  [wrist_R] -> Joint Actuator7/1
  [wrist_L] -> Gain2/1
  [wrist_L] -> Gain3/1
  [wrist_L] -> Gain4/1
  Shoulders/1 -> [Flapping]
  Teta1_R/1 -> [Humerus_R]
  Teta1_L/1 -> [Humerus_L]
  elbow_R/1 -> [Radius_R]
  elbow_L/1 -> [Radius_L]
  wrist_R/1 -> [wrist_R]
  wrist_L/1 -> [wrist_L]
  Gain/1 -> Joint Actuator5/1
  [wrist_R] -> Gain/1
  Gain1/1 -> Joint Actuator6/1
  Gain3/1 -> Joint Actuator9/1
  Gain4/1 -> Joint Actuator10/1
  Gain2/1 -> Joint Actuator8/1
  Constant2/1 -> Motion Driver With Displacement Input1/1
  [legs] -> Joint Actuator11/1
  [legs] -> Joint Actuator12/1
  Motion Driver With Displacement Input1/1 -> [legs]
  Flapping/1 -> [F_p]
  Flapping/2 -> [F_R]
  [F_R] -> Flapping_Angle/1
  [HL_R] -> HumerusLEFT_Angle/1
  [RL_R] -> RadiusLEFT_Angle/1
  [HR_R] -> HumerusRIGHT_Angle/1
  [RR_R] -> RadiusRIGHT_Angle/1
  [fb_p] -> Base_POS/1
  [fb_R] -> Base_Angles/1
  connections:
  barra_servo-1/RConn1 -- Cylindrical/LConn1
  Cylindrical/RConn1 -- barra5-1/LConn2
  body5_2_right-1/RConn3 -- Cylindrical1/LConn1
  Cylindrical1/RConn1 -- motor_case-2/LConn2
  barra_servo-1/RConn2 -- Cylindrical2/LConn1
  Cylindrical2/RConn1 -- barra5-2/LConn2
  RootGround/LConn1 -- Machine Environment/RConn1
  body5_2_left-1/RConn2 -- Prismatic/LConn1
  Prismatic/RConn1 -- motor_case-2/LConn1
  Revolute/RConn1 -- barra_servo-1/LConn1
  shoulder5_right-1/RConn1 -- Revolute1/LConn1
  Revolute1/RConn1 -- barra5-1/LConn1
  humerus5_left-1/RConn1 -- Revolute10/LConn1
  Revolute10/RConn1 -- radius5-2/LConn1
  radius5-1/RConn1 -- Revolute11/LConn1
  Revolute11/RConn1 -- digit 5-1/LConn1
  digit 5-1/RConn1 -- Revolute12/LConn1
  Revolute12/RConn1 -- digit 4-1/LConn1
  radius5-2/RConn1 -- Revolute13/LConn1
  Revolute13/RConn1 -- digit 5-2/LConn1
  radius5-2/RConn2 -- Revolute14/LConn1
  Revolute14/RConn1 -- digit 3-2/LConn1
  digit 5-2/RConn1 -- Revolute15/LConn1
  Revolute15/RConn1 -- digit 4-2/LConn1
  radius5-1/RConn2 -- Revolute16/LConn1
  Revolute16/RConn1 -- digit 3-1/LConn1
  body5_2_left-1/RConn1 -- Revolute2/LConn1
  Revolute2/RConn1 -- shoulder5_left-1/LConn1
  shoulder5_left-1/RConn1 -- Revolute3/LConn1
  Revolute3/RConn1 -- humerus5_left-1/LConn1
  shoulder5_left-1/RConn2 -- Revolute4/LConn1
  Revolute4/RConn1 -- barra5-2/LConn1
  body5_2_right-1/RConn1 -- Revolute5/LConn1
  Revolute5/RConn1 -- shoulder5_right-1/LConn1
  shoulder5_right-1/RConn2 -- Revolute6/LConn1
  Revolute6/RConn1 -- humerus5_right-1/LConn1
  body5_2_left-1/RConn3 -- Revolute7/LConn1
  Revolute7/RConn1 -- leg-2/LConn1
  body5_2_right-1/RConn4 -- Revolute8/LConn1
  Revolute8/RConn1 -- leg-1/LConn1
  humerus5_right-1/RConn1 -- Revolute9/LConn1
  Revolute9/RConn1 -- radius5-1/LConn1
  RootGround/RConn1 -- Six-DoF/LConn1
  Six-DoF/RConn1 -- RootPart/LConn1
  RootPart/RConn1 -- Weld/LConn1
  Weld/RConn1 -- body5_2_right-1/LConn1
  motor_case-2/RConn1 -- Weld1/LConn1
  Weld1/RConn1 -- servo-1/LConn1
  body5_2_right-1/RConn2 -- Weld2/LConn1
  Weld2/RConn1 -- body5_2_left-1/LConn1
  Floating-base/LConn1 -- RootPart/RConn2
  shoulder-right/LConn1 -- shoulder5_right-1/RConn3
  shoulder-left/LConn1 -- shoulder5_left-1/RConn3
  humerus-left/LConn1 -- humerus5_left-1/RConn2
  humerus-right/LConn1 -- humerus5_right-1/RConn2
  radius-left/LConn1 -- radius5-2/RConn3
  radius-right/LConn1 -- radius5-1/RConn3
  digit5-1/LConn1 -- digit 5-1/RConn2
  digit3-1/LConn1 -- digit 3-1/RConn1
  digit 4-1/RConn1 -- digit4-1/LConn1
  digit5-2/LConn1 -- digit 5-2/RConn2
  digit3-2/LConn1 -- digit 3-2/RConn1
  digit4-2/LConn1 -- digit 4-2/RConn1
  Joint Actuator/RConn1 -- Revolute/LConn2
  Revolute3/LConn2 -- Joint Actuator2/RConn1
  Joint Actuator3/RConn1 -- Revolute10/LConn2
  Revolute9/LConn2 -- Joint Actuator4/RConn1
  Joint Actuator1/RConn1 -- Revolute6/LConn2
  servo-1/RConn1 -- Revolute/LConn1
  Joint Actuator5/RConn1 -- Revolute11/LConn2
  Revolute12/LConn2 -- Joint Actuator6/RConn1
  Joint Actuator7/RConn1 -- Revolute16/LConn2
  Joint Actuator8/RConn1 -- Revolute13/LConn2
  Joint Actuator9/RConn1 -- Revolute15/LConn2
  Revolute14/LConn2 -- Joint Actuator10/RConn1
  Joint Actuator11/RConn1 -- Revolute8/LConn2
  Joint Actuator12/RConn1 -- Revolute7/LConn2
  Flapping/LConn1 -- barra_servo-1/RConn3
